simulink model "ElevatorPlant_Storage_A"  (R2015b)
(part 7 of 8)

            (junction 94133) -> Emergency.Doors.Opening2.Button_detection1.BUTTON_CAR.Button_CAR_1 [order 1] : [P1]
            (junction 94133) -> (junction 94134) [order 2]
            (junction 94135) -> (junction 94134)
            (junction 94136) -> (junction 94135)
            (junction 94134) -> (junction 94137)
            (junction 94137) -> Emergency.Doors.Opening2.Button_detection1.BUTTON_CAR.Button_CAR_2 [order 1] : [P2]
            Emergency.Doors.Opening2.Button_detection1.BUTTON_CAR.Button_CAR_2 -> (junction 94138)
            (junction 94138) -> Emergency.Doors.Opening2.Button_detection1.BUTTON_CAR.First_but_2 [order 1] : [FIRST_BUT && not(RPC2)]
            Emergency.Doors.Opening2.Button_detection1.BUTTON_CAR.First_but_2 -> (junction 94139)
            (junction 94137) -> (junction 94140) [order 2]
            (junction 94138) -> (junction 94141) [order 2]
            (junction 94139) -> (junction 94142)
            (junction 94141) -> (junction 94140)
            (junction 94142) -> (junction 94141)
            (junction 94140) -> (junction 94143)
            (junction 94143) -> Emergency.Doors.Opening2.Button_detection1.BUTTON_CAR.Button_CAR_3 [order 1] : [P3]
            Emergency.Doors.Opening2.Button_detection1.BUTTON_CAR.Button_CAR_3 -> (junction 94144)
            (junction 94144) -> Emergency.Doors.Opening2.Button_detection1.BUTTON_CAR.First_but_3 [order 1] : [FIRST_BUT && not(RPC3)]
            Emergency.Doors.Opening2.Button_detection1.BUTTON_CAR.First_but_3 -> (junction 94145)
            (junction 94143) -> (junction 94146) [order 2]
            (junction 94144) -> (junction 94147) [order 2]
            (junction 94145) -> (junction 94148)
            (junction 94147) -> (junction 94146)
            (junction 94148) -> (junction 94147)
          state BUTTON_UP
            state Button_UP_0
              en:
              BUTTON_UP(1)=true;
              BUT_TEMP=0;
              LPS0=true;
              PUSHED=true;
              UPDATE=false;
              IN_LL=false; ET_LL=0;
            state First_but_0
              en:
              BUT_1=BUT_TEMP;
              FIRST_BUT=false;
            state Button_UP_1
              en:
              BUTTON_UP(2)=true;
              BUT_TEMP=1;
              LPS1=true;
              PUSHED=true;
              UPDATE=false;
              IN_LL=false; ET_LL=0;
            state First_but_1
              en:
              BUT_1=BUT_TEMP;
              FIRST_BUT=false;
            state Button_UP_2
              en:
              BUTTON_UP(3)=true;
              BUT_TEMP=2;
              LPS2=true;
              PUSHED=true;
              UPDATE=false;
              IN_LL=false; ET_LL=0;
            state First_but_2
              en:
              BUT_1=BUT_TEMP;
              FIRST_BUT=false;
            (junction 94198) -> Emergency.Doors.Opening2.Button_detection1.BUTTON_UP.Button_UP_0 [order 1] : [PS0]
            Emergency.Doors.Opening2.Button_detection1.BUTTON_UP.Button_UP_0 -> (junction 94199)
            (junction 94199) -> Emergency.Doors.Opening2.Button_detection1.BUTTON_UP.First_but_0 [order 1] : [FIRST_BUT && not(RPC0)]
            Emergency.Doors.Opening2.Button_detection1.BUTTON_UP.First_but_0 -> (junction 94200)
            (default) -> (junction 94198)
            (junction 94198) -> (junction 94203) [order 2]
            (junction 94199) -> (junction 94201) [order 2]
            (junction 94200) -> (junction 94202)
            (junction 94202) -> (junction 94201)
            (junction 94201) -> (junction 94203)
            (junction 94203) -> (junction 94204)
            (junction 94204) -> Emergency.Doors.Opening2.Button_detection1.BUTTON_UP.Button_UP_1 [order 1] : [PS1]
            Emergency.Doors.Opening2.Button_detection1.BUTTON_UP.Button_UP_1 -> (junction 94205)
            (junction 94205) -> Emergency.Doors.Opening2.Button_detection1.BUTTON_UP.First_but_1 [order 1] : [FIRST_BUT && not(RPC1)]
            Emergency.Doors.Opening2.Button_detection1.BUTTON_UP.First_but_1 -> (junction 94206)
            (junction 94204) -> (junction 94207) [order 2]
            (junction 94205) -> (junction 94208) [order 2]
            (junction 94206) -> (junction 94209)
            (junction 94208) -> (junction 94207)
            (junction 94209) -> (junction 94208)
            (junction 94207) -> (junction 94211)
            Emergency.Doors.Opening2.Button_detection1.BUTTON_UP.First_but_2 -> (junction 94210)
            (junction 94210) -> (junction 94215)
            (junction 94211) -> Emergency.Doors.Opening2.Button_detection1.BUTTON_UP.Button_UP_2 [order 1] : [PS2]
            Emergency.Doors.Opening2.Button_detection1.BUTTON_UP.Button_UP_2 -> (junction 94212)
            (junction 94212) -> Emergency.Doors.Opening2.Button_detection1.BUTTON_UP.First_but_2 [order 1] : [FIRST_BUT && not(RPC2)]
            (junction 94211) -> (junction 94213) [order 2]
            (junction 94212) -> (junction 94214) [order 2]
            (junction 94214) -> (junction 94213)
            (junction 94215) -> (junction 94214)
          state Max_Min_assignment
            state Min_but
              en:
              BUTTON=MIN_BUT;
            state Max_but
              en:
              BUTTON=MAX_BUT;
            state First_but
              en:
              BUTTON=BUT_1;
            state Max_but1
              en:
              MAX_BUT=2;
            state Max_but2
              en:
              MAX_BUT=1;
            state Max_but3
              en:
              MAX_BUT=0;
            state Min_but1
              en:
              MIN_BUT=1;
            state Min_but2
              en:
              MIN_BUT=2;
            state Min_but3
              en:
              MIN_BUT=3;
            state MAX
              en:
              MAX_BUT=BUT_TEMP;
            state MIN
              en:
              MIN_BUT=BUT_TEMP;
            state Updating_button_0
              en:
              BUTTON=MAX_BUT;
            state Updating_button_1
              en:
              BUTTON=MIN_BUT;
            (junction 94253) -> Emergency.Doors.Opening2.Button_detection1.Max_Min_assignment.Min_but [order 1] : [(MAX_BUT-FLOOR)>(FLOOR-MIN_BUT)]
            Emergency.Doors.Opening2.Button_detection1.Max_Min_assignment.Min_but -> (junction 94254)
            (junction 94255) -> (junction 94253) [order 1] : [not(FLAG_STOP) && MOTION==2 && FLAG==3]
            (default) -> (junction 94255)
            (junction 94253) -> (junction 94256) [order 2]
            (junction 94254) -> (junction 94257)
            (junction 94255) -> (junction 94258) [order 2]
            (junction 94256) -> Emergency.Doors.Opening2.Button_detection1.Max_Min_assignment.Max_but [order 1] : [(MAX_BUT-FLOOR)<(FLOOR-MIN_BUT)]
            Emergency.Doors.Opening2.Button_detection1.Max_Min_assignment.Max_but -> (junction 94257)
            (junction 94256) -> Emergency.Doors.Opening2.Button_detection1.Max_Min_assignment.First_but [order 2]
            (junction 94257) -> (junction 94260)
            Emergency.Doors.Opening2.Button_detection1.Max_Min_assignment.First_but -> (junction 94259)
            (junction 94259) -> (junction 94258)
            (junction 94260) -> (junction 94259)
            (junction 94258) -> (junction 94261)
            (junction 94262) -> (junction 94263) [order 1] : [MOTION==0]
                | {MOTION=1;
                | UPDATE=true;}
            (junction 94263) -> Emergency.Doors.Opening2.Button_detection1.Max_Min_assignment.Max_but1 [order 1] : [BUTTON_UP(2)]
            Emergency.Doors.Opening2.Button_detection1.Max_Min_assignment.Max_but1 -> (junction 94264)
            (junction 94261) -> (junction 94262) [order 1] : [BUTTON==FLOOR && EXTEND]
                | {EXTEND=false;}
            (junction 94261) -> (junction 94275) [order 2]
            (junction 94262) -> (junction 94267) [order 2]
            (junction 94263) -> (junction 94265) [order 2]
            (junction 94264) -> (junction 94266)
            (junction 94265) -> Emergency.Doors.Opening2.Button_detection1.Max_Min_assignment.Max_but2 [order 1] : [BUTTON_UP(1)]
            Emergency.Doors.Opening2.Button_detection1.Max_Min_assignment.Max_but2 -> (junction 94266)
            (junction 94265) -> Emergency.Doors.Opening2.Button_detection1.Max_Min_assignment.Max_but3 [order 2]
            (junction 94266) -> (junction 94269)
            Emergency.Doors.Opening2.Button_detection1.Max_Min_assignment.Max_but3 -> (junction 94268)
            (junction 94268) -> (junction 94267)
            (junction 94269) -> (junction 94268)
            (junction 94267) -> (junction 94270)
            (junction 94270) -> (junction 94271) [order 1] : [MOTION==1]
                | {MOTION=0;
                | UPDATE=true;}
            (junction 94271) -> Emergency.Doors.Opening2.Button_detection1.Max_Min_assignment.Min_but1 [order 1] : [BUTTON_DOWN(1)]
            Emergency.Doors.Opening2.Button_detection1.Max_Min_assignment.Min_but1 -> (junction 94272)
            (junction 94270) -> (junction 94276) [order 2]
            (junction 94271) -> (junction 94273) [order 2]
            (junction 94272) -> (junction 94274)
            (junction 94273) -> Emergency.Doors.Opening2.Button_detection1.Max_Min_assignment.Min_but2 [order 1] : [BUTTON_DOWN(2)]
            Emergency.Doors.Opening2.Button_detection1.Max_Min_assignment.Min_but2 -> (junction 94274)
            (junction 94273) -> Emergency.Doors.Opening2.Button_detection1.Max_Min_assignment.Min_but3 [order 2]
            (junction 94274) -> (junction 94278)
            Emergency.Doors.Opening2.Button_detection1.Max_Min_assignment.Min_but3 -> (junction 94277)
            (junction 94276) -> (junction 94275)
            (junction 94277) -> (junction 94276)
            (junction 94278) -> (junction 94277)
            (junction 94275) -> (junction 94280)
            Emergency.Doors.Opening2.Button_detection1.Max_Min_assignment.MAX -> (junction 94279)
            (junction 94280) -> (junction 94281) [order 1] : [PUSHED]
            (junction 94281) -> (junction 94282) [order 1] : [not(BUT_TEMP==FLOOR) || not(MOTION==2)]
            (junction 94282) -> Emergency.Doors.Opening2.Button_detection1.Max_Min_assignment.MAX [order 1] : [MAX_BUT<BUT_TEMP && not(UPDATE)]
            (junction 94279) -> (junction 94284)
            (junction 94280) -> (junction 94294) [order 2]
            (junction 94281) -> (junction 94287) [order 2]
            (junction 94282) -> (junction 94283) [order 2]
            (junction 94284) -> (junction 94283)
            (junction 94283) -> (junction 94285)
            (junction 94285) -> Emergency.Doors.Opening2.Button_detection1.Max_Min_assignment.MIN [order 1] : [MIN_BUT>BUT_TEMP && not(UPDATE)]
            Emergency.Doors.Opening2.Button_detection1.Max_Min_assignment.MIN -> (junction 94286)
            (junction 94285) -> (junction 94288) [order 2]
            (junction 94286) -> (junction 94289)
            (junction 94288) -> (junction 94287)
            (junction 94289) -> (junction 94288)
            (junction 94287) -> (junction 94290)
            (junction 94290) -> Emergency.Doors.Opening2.Button_detection1.Max_Min_assignment.Updating_button_0 [order 1] : [MOTION==0]
            Emergency.Doors.Opening2.Button_detection1.Max_Min_assignment.Updating_button_0 -> (junction 94291)
            (junction 94290) -> (junction 94292) [order 2]
            (junction 94291) -> (junction 94293)
            (junction 94292) -> Emergency.Doors.Opening2.Button_detection1.Max_Min_assignment.Updating_button_1 [order 1] : [MOTION==1]
            Emergency.Doors.Opening2.Button_detection1.Max_Min_assignment.Updating_button_1 -> (junction 94293)
            (junction 94292) -> (junction 94295) [order 2]
            (junction 94293) -> (junction 94296)
            (junction 94295) -> (junction 94294)
            (junction 94296) -> (junction 94295)
          state GoTo_PositionControl
            en:
            BUTTON=BUT_TEMP;
            FLAG=2;
          state Emergency
            en:
            FLAG_EMG=true;
            FLAG=4;
          state Timer_EME
            state Set_tmr
              en:
              Q_EME=true;
            state Counting
              en:
              ET_EME= ET_EME + 1;
              Q_EME=false;
            state Set
              en:
              IN_EME=true;
              PT_EME=3;
            (junction 94386) -> Emergency.Doors.Opening2.Button_detection1.Timer_EME.Set_tmr [order 1] : [ET_EME==PT_EME]
            Emergency.Doors.Opening2.Button_detection1.Timer_EME.Set_tmr -> (junction 94387)
            Emergency.Doors.Opening2.Button_detection1.Timer_EME.Counting -> (junction 94386)
            (junction 94386) -> (junction 94387) [order 2]
            (default) -> Emergency.Doors.Opening2.Button_detection1.Timer_EME.Set
            Emergency.Doors.Opening2.Button_detection1.Timer_EME.Set -> (junction 94388)
            (junction 94388) -> Emergency.Doors.Opening2.Button_detection1.Timer_EME.Counting [order 1] : [ET_EME<PT_EME]
            (junction 94388) -> (junction 94387) [order 2]
          state Not_Emergency
            en:
            IN_EME=false;
            ET_EME=0;
          state SwitchingOFF_LEDs
            en:
            LPD3=false;
            LPD2=false;
            LPS2=false;
            LPD1=false;
            LPS1=false;
            LPS0=false;
          (default) -> (junction 93987)
          (junction 93987) -> (junction 93988) [order 1] : [FLAG==1 && not(PUSHED)]
              | {BUTTON=FLOOR;
              | BUT_TEMP=BUTTON;
              | BUT_1=FLOOR;}
          (junction 93988) -> Emergency.Doors.Opening2.Button_detection1.Timer_LL [order 1] : [not(FLAG_STOP)]
          Emergency.Doors.Opening2.Button_detection1.Save_energy -> (junction 93989)
          Emergency.Doors.Opening2.Button_detection1.Timer_LL -> Emergency.Doors.Opening2.Button_detection1.Save_energy
          (junction 93988) -> (junction 93991) [order 2]
          (junction 93987) -> (junction 93990) [order 2]
          (junction 93989) -> (junction 93992)
          (junction 93991) -> (junction 93990)
          (junction 93992) -> (junction 93991)
          (junction 93990) -> Emergency.Doors.Opening2.Button_detection1.BUTTON_CAR
          Emergency.Doors.Opening2.Button_detection1.BUTTON_UP -> Emergency.Doors.Opening2.Button_detection1.BUTTON_DOWN
          Emergency.Doors.Opening2.Button_detection1.BUTTON_DOWN -> Emergency.Doors.Opening2.Button_detection1.Max_Min_assignment
          Emergency.Doors.Opening2.Button_detection1.Max_Min_assignment -> (junction 93993)
          Emergency.Doors.Opening2.Button_detection1.BUTTON_CAR -> Emergency.Doors.Opening2.Button_detection1.BUTTON_UP
          (junction 93993) -> (junction 93995)
          (junction 93995) -> (junction 93994)
          (junction 93994) -> (junction 93997)
          Emergency.Doors.Opening2.Button_detection1.GoTo_PositionControl -> (junction 93996)
          (junction 93997) -> (junction 93998) [order 1] : [FLAG==1]
          (junction 93998) -> Emergency.Doors.Opening2.Button_detection1.GoTo_PositionControl [order 1] : [PUSHED]
          (junction 93996) -> (junction 94000)
          (junction 93997) -> (junction 94008) [order 2]
          (junction 93998) -> (junction 93999) [order 2]
          (junction 94000) -> (junction 93999)
          (junction 93999) -> (junction 94002)
          Emergency.Doors.Opening2.Button_detection1.Emergency -> (junction 94001)
          (junction 94002) -> Emergency.Doors.Opening2.Button_detection1.Timer_EME [order 1] : [STOP]
              | {IN_LL=false; ET_LL=0;FLAG=1;}
          Emergency.Doors.Opening2.Button_detection1.Timer_EME -> (junction 94003)
          (junction 94003) -> Emergency.Doors.Opening2.Button_detection1.Emergency [order 1] : [Q_EME]
          (junction 94001) -> (junction 94005)
          (junction 94002) -> Emergency.Doors.Opening2.Button_detection1.Not_Emergency [order 2]
          (junction 94003) -> (junction 94004) [order 2]
          (junction 94005) -> (junction 94004)
          (junction 94004) -> (junction 94007)
          Emergency.Doors.Opening2.Button_detection1.Not_Emergency -> (junction 94007)
          Emergency.Doors.Opening2.Button_detection1.SwitchingOFF_LEDs -> (junction 94006)
          (junction 94007) -> Emergency.Doors.Opening2.Button_detection1.SwitchingOFF_LEDs [order 1] : [FLAG_STOP && FLAG==2]
          (junction 94006) -> (junction 94010)
          (junction 94007) -> (junction 94009) [order 2]
          (junction 94009) -> (junction 94008)
          (junction 94010) -> (junction 94009)
        state Opening1
          en:AP2=true;
        state Reset
          state Reset_0
            en:
            LPS0=false;
            BUTTON_CAR(1)=false;
            BUTTON_UP(1)=false;
          state Reset_1
            en:
            LPS1=false;
            LPD1=false;
            BUTTON_CAR(2)=false;
            BUTTON_UP(2)=false;
            BUTTON_DOWN(2)=false;
          state Reset_2
            en:
            LPS2=false;
            LPD2=false;
            BUTTON_CAR(3)=false;
            BUTTON_UP(3)=false;
            BUTTON_DOWN(3)=false;
          state Reset_3
            en:
            LPD3=false;
            BUTTON_CAR(4)=false;
            BUTTON_DOWN(4)=false;
          (default) -> (junction 94404)
          (junction 94404) -> Emergency.Doors.Opening2.Reset.Reset_0 [order 1] : [FLOOR==0]
          Emergency.Doors.Opening2.Reset.Reset_0 -> (junction 94405)
          (junction 94404) -> (junction 94406) [order 2]
          (junction 94405) -> (junction 94407)
          (junction 94406) -> Emergency.Doors.Opening2.Reset.Reset_1 [order 1] : [FLOOR==1]
          Emergency.Doors.Opening2.Reset.Reset_1 -> (junction 94407)
          (junction 94406) -> (junction 94408) [order 2]
          (junction 94407) -> (junction 94409)
          (junction 94408) -> Emergency.Doors.Opening2.Reset.Reset_2 [order 1] : [FLOOR==2]
          Emergency.Doors.Opening2.Reset.Reset_2 -> (junction 94409)
          (junction 94408) -> (junction 94410) [order 2]
          (junction 94409) -> (junction 94411)
          (junction 94410) -> Emergency.Doors.Opening2.Reset.Reset_3 [order 1] : [FLOOR==3]
          Emergency.Doors.Opening2.Reset.Reset_3 -> (junction 94411)
          (junction 94410) -> (junction 94412) [order 2]
          (junction 94411) -> (junction 94413)
          (junction 94413) -> (junction 94412)
        state Stop_Opening1
          en: AP2=false;
          FLAG_OD=true;
          IN_cl=false;
          ET_cl=0;
        (junction 93401) -> (junction 93402)
        (junction 93402) -> (junction 93403) [order 1] : [not(OBS) ]
        (junction 93405) -> Emergency.Doors.Opening2.Opening [order 1] : [not(PA2)]
        (junction 93403) -> (junction 93404) [order 2]
        (junction 93404) -> Emergency.Doors.Opening2.Timer_open
        Emergency.Doors.Opening2.Timer_open -> (junction 93405)
        (default) -> Emergency.Doors.Opening2.People_IN
        (junction 93402) -> (junction 93406) [order 2]
        (junction 93403) -> Emergency.Doors.Opening2.Button_detection [order 1] : [not(FLAG==4)]
        (junction 93408) -> (junction 93404)
        (junction 93410) -> (junction 93401)
        (junction 93405) -> Emergency.Doors.Opening2.Stop_Opening [order 2]
        Emergency.Doors.Opening2.People_IN -> Emergency.Doors.Opening2.People_OUT
        Emergency.Doors.Opening2.Opening -> (junction 93415)
        (junction 93406) -> (junction 93407) [order 2]
        (junction 93406) -> Emergency.Doors.Opening2.Button_detection1 [order 1] : [not(FLAG==4)]
        (junction 93407) -> (junction 93412)
        Emergency.Doors.Opening2.Button_detection -> (junction 93408)
        Emergency.Doors.Opening2.People_OUT -> (junction 93409)
        Emergency.Doors.Opening2.Button_detection1 -> (junction 93411)
        (junction 93412) -> (junction 93411)
        (junction 93409) -> (junction 93410) [order 2]
        (junction 93409) -> Emergency.Doors.Opening2.Reset [order 1] : [not(FLAG==4)]
        (junction 93411) -> (junction 93413)
        (junction 93419) -> (junction 93410)
        Emergency.Doors.Opening2.Stop_Opening -> (junction 93414)
        (junction 93413) -> Emergency.Doors.Opening2.Opening1 [order 1] : [not(PA2)]
        (junction 93413) -> Emergency.Doors.Opening2.Stop_Opening1 [order 2]
        (junction 93415) -> (junction 93414)
        (junction 93414) -> (junction 93417)
        Emergency.Doors.Opening2.Opening1 -> (junction 93416)
        Emergency.Doors.Opening2.Reset -> (junction 93418)
        Emergency.Doors.Opening2.Stop_Opening1 -> (junction 93416)
        (junction 93416) -> (junction 93417)
        (junction 93418) -> (junction 93419)
      state FLOOR_3
        en: CP3=false;
      state Opening3
        state Opening
          en:AP3=Q_op;
        state People_IN
          state Check_People_IN
            en:
            COUNTER_IN=false;
          state People_KID_IN
            en:
            WEIGHT=WEIGHT+30;
            KIDS=KIDS+1;
          state People_WOMAN_IN
            en:
            WEIGHT=WEIGHT+55;
            WOMEN=WOMEN+1;
          state People_MAN_IN
            en:
            WEIGHT=WEIGHT+75;
            MEN=MEN+1;
          state People_FATGUY_IN
            en:
            WEIGHT=WEIGHT+100;
            FATGUYS=FATGUYS+1;
          state Re_Ready_IN
            en:
            COUNTER_IN=true;
          (default) -> (junction 94494)
          (junction 94494) -> Emergency.Doors.Opening3.People_IN.Check_People_IN [order 1] : [COUNTER_IN]
          Emergency.Doors.Opening3.People_IN.Check_People_IN -> (junction 94495)
          (junction 94495) -> Emergency.Doors.Opening3.People_IN.People_KID_IN [order 1] : [KID_IN]
          Emergency.Doors.Opening3.People_IN.People_KID_IN -> (junction 94496)
          (junction 94494) -> (junction 94503) [order 2]
          (junction 94495) -> (junction 94497) [order 2]
          (junction 94496) -> (junction 94498)
          (junction 94497) -> Emergency.Doors.Opening3.People_IN.People_WOMAN_IN [order 1] : [WOMAN_IN]
          Emergency.Doors.Opening3.People_IN.People_WOMAN_IN -> (junction 94498)
          (junction 94497) -> (junction 94499) [order 2]
          (junction 94498) -> (junction 94500)
          (junction 94499) -> Emergency.Doors.Opening3.People_IN.People_MAN_IN [order 1] : [MAN_IN]
          Emergency.Doors.Opening3.People_IN.People_MAN_IN -> (junction 94500)
          (junction 94499) -> (junction 94501) [order 2]
          (junction 94500) -> (junction 94502)
          (junction 94501) -> Emergency.Doors.Opening3.People_IN.People_FATGUY_IN [order 1] : [FATGUY_IN]
          Emergency.Doors.Opening3.People_IN.People_FATGUY_IN -> (junction 94502)
          (junction 94501) -> (junction 94504) [order 2]
          (junction 94502) -> (junction 94505)
          (junction 94504) -> (junction 94503)
          (junction 94505) -> (junction 94504)
          (junction 94503) -> (junction 94506)
          (junction 94506) -> Emergency.Doors.Opening3.People_IN.Re_Ready_IN [order 1] : [not(KID_IN|| WOMAN_IN || MAN_IN || FATGUY_IN)]
          (junction 94506) -> (junction 94507) [order 2]
          Emergency.Doors.Opening3.People_IN.Re_Ready_IN -> (junction 94508)
          (junction 94508) -> (junction 94507)
        state Timer_open
          state Set_tmr
            en: Q_op=true;
          state Set
            en:PT_op=2;
            IN_op=true;
          state Counting
            en:ET_op = ET_op + 1;
            Q_op=false;
          (junction 94543) -> Emergency.Doors.Opening3.Timer_open.Set_tmr [order 1] : [ET_op==PT_op]
          Emergency.Doors.Opening3.Timer_open.Set_tmr -> (junction 94544)
          (default) -> Emergency.Doors.Opening3.Timer_open.Set
          Emergency.Doors.Opening3.Timer_open.Counting -> (junction 94543)
          (junction 94543) -> (junction 94544) [order 2]
          Emergency.Doors.Opening3.Timer_open.Set -> (junction 94545)
          (junction 94545) -> Emergency.Doors.Opening3.Timer_open.Counting [order 1] : [ET_op<PT_op]
          (junction 94545) -> (junction 94544) [order 2]
        state Stop_Opening
          en:AP3=false;
          FLAG_OD=true;
          OBS=true;
          IN_op=false;
          ET_op=0;
        state People_OUT
          state Check_People_OUT
            en:
            COUNTER_OUT=false;
          state People_KID_OUT
            en:
            WEIGHT=WEIGHT-30;
            KIDS=KIDS-1;
          state People_WOMAN_OUT
            en:
            WEIGHT=WEIGHT-55;
            WOMEN=WOMEN-1;
          state People_MAN_OUT
            en:
            WEIGHT=WEIGHT-75;
            MEN=MEN-1;
          state People_FATGUY_OUT
            en:
            WEIGHT=WEIGHT-100;
            FATGUYS=FATGUYS-1;
          state Re_Ready_OUT
            en:
            COUNTER_OUT=true;
          (default) -> (junction 94559)
          (junction 94559) -> Emergency.Doors.Opening3.People_OUT.Check_People_OUT [order 1] : [COUNTER_OUT]
          Emergency.Doors.Opening3.People_OUT.Check_People_OUT -> (junction 94560)
          (junction 94560) -> Emergency.Doors.Opening3.People_OUT.People_KID_OUT [order 1] : [KID_OUT && KIDS>0 ]
          Emergency.Doors.Opening3.People_OUT.People_KID_OUT -> (junction 94561)
          (junction 94559) -> (junction 94568) [order 2]
          (junction 94560) -> (junction 94562) [order 2]
          (junction 94561) -> (junction 94563)
          (junction 94562) -> Emergency.Doors.Opening3.People_OUT.People_WOMAN_OUT [order 1] : [WOMAN_OUT && WOMEN>0]
          Emergency.Doors.Opening3.People_OUT.People_WOMAN_OUT -> (junction 94563)
          (junction 94563) -> (junction 94565)
          (junction 94562) -> (junction 94564) [order 2]
          (junction 94564) -> Emergency.Doors.Opening3.People_OUT.People_MAN_OUT [order 1] : [MAN_OUT && MEN>0]
          Emergency.Doors.Opening3.People_OUT.People_MAN_OUT -> (junction 94565)
          (junction 94564) -> (junction 94566) [order 2]
          (junction 94565) -> (junction 94567)
          (junction 94566) -> Emergency.Doors.Opening3.People_OUT.People_FATGUY_OUT [order 1] : [FATGUY_OUT && FATGUYS>0]
          Emergency.Doors.Opening3.People_OUT.People_FATGUY_OUT -> (junction 94567)
          (junction 94566) -> (junction 94569) [order 2]
          (junction 94567) -> (junction 94570)
          (junction 94569) -> (junction 94568)
          (junction 94570) -> (junction 94569)
          (junction 94568) -> (junction 94571)
          (junction 94571) -> Emergency.Doors.Opening3.People_OUT.Re_Ready_OUT [order 1] : [not(KID_OUT || WOMAN_OUT || MAN_OUT || FATGUY_OUT)]
          (junction 94571) -> (junction 94572) [order 2]
          Emergency.Doors.Opening3.People_OUT.Re_Ready_OUT -> (junction 94573)
          (junction 94573) -> (junction 94572)
        state Button_detection
          state Save_energy
            en:
            LL=not(Q_LL);
          state Timer_LL
            state Set_tmr
              en:
              Q_LL=true;
            state Counting
              en:
              ET_LL= ET_LL + 1;
              Q_LL=false;
            state Set
              en:
              IN_LL=true;
              PT_LL=10;
            (junction 94676) -> Emergency.Doors.Opening3.Button_detection.Timer_LL.Set_tmr [order 1] : [ET_LL==PT_LL]
            Emergency.Doors.Opening3.Button_detection.Timer_LL.Set_tmr -> (junction 94677)
            Emergency.Doors.Opening3.Button_detection.Timer_LL.Counting -> (junction 94676)
            (junction 94676) -> (junction 94677) [order 2]
            (default) -> Emergency.Doors.Opening3.Button_detection.Timer_LL.Set
            Emergency.Doors.Opening3.Button_detection.Timer_LL.Set -> (junction 94678)
            (junction 94678) -> Emergency.Doors.Opening3.Button_detection.Timer_LL.Counting [order 1] : [ET_LL<PT_LL]
            (junction 94678) -> (junction 94677) [order 2]
          state BUTTON_DOWN
            state Button_DOWN_1
              en:
              BUTTON_DOWN(2)=true;
              BUT_TEMP=1;
              LPD1=true;
              PUSHED=true;
              UPDATE=false;
              IN_LL=false; ET_LL=0;
            state First_but_1
              en:
              BUT_1=BUT_TEMP;
              FIRST_BUT=false;
            state Button_DOWN_2
              en:
              BUTTON_DOWN(3)=true;
              BUT_TEMP=2;
              LPD2=true;
              PUSHED=true;
              UPDATE=false;
              IN_LL=false; ET_LL=0;
            state First_but_2
              en:
              BUT_1=BUT_TEMP;
              FIRST_BUT=false;
            state Button_DOWN_3
              en:
              BUTTON_DOWN(4)=true;
              BUT_TEMP=3;
              LPD3=true;
              PUSHED=true;
              UPDATE=false;
              IN_LL=false; ET_LL=0;
            state First_but_3
              en:
              BUT_1=BUT_TEMP;
              FIRST_BUT=false;
            (default) -> (junction 94691)
            (junction 94691) -> Emergency.Doors.Opening3.Button_detection.BUTTON_DOWN.Button_DOWN_1 [order 1] : [PD1]
            Emergency.Doors.Opening3.Button_detection.BUTTON_DOWN.Button_DOWN_1 -> (junction 94692)
            (junction 94692) -> Emergency.Doors.Opening3.Button_detection.BUTTON_DOWN.First_but_1 [order 1] : [FIRST_BUT && not(RPC1)]
            Emergency.Doors.Opening3.Button_detection.BUTTON_DOWN.First_but_1 -> (junction 94693)
            (junction 94691) -> (junction 94694) [order 2]
            (junction 94692) -> (junction 94695) [order 2]
            (junction 94693) -> (junction 94696)
            (junction 94695) -> (junction 94694)
            (junction 94696) -> (junction 94695)
            (junction 94694) -> (junction 94697)
            (junction 94697) -> Emergency.Doors.Opening3.Button_detection.BUTTON_DOWN.Button_DOWN_2 [order 1] : [PD2]
            Emergency.Doors.Opening3.Button_detection.BUTTON_DOWN.Button_DOWN_2 -> (junction 94698)
            (junction 94698) -> Emergency.Doors.Opening3.Button_detection.BUTTON_DOWN.First_but_2 [order 1] : [FIRST_BUT && not(RPC2)]
            Emergency.Doors.Opening3.Button_detection.BUTTON_DOWN.First_but_2 -> (junction 94699)
            (junction 94697) -> (junction 94700) [order 2]
            (junction 94698) -> (junction 94701) [order 2]
            (junction 94699) -> (junction 94702)
            (junction 94701) -> (junction 94700)
            (junction 94702) -> (junction 94701)
            (junction 94700) -> (junction 94703)
            (junction 94703) -> Emergency.Doors.Opening3.Button_detection.BUTTON_DOWN.Button_DOWN_3 [order 1] : [PD3]
            Emergency.Doors.Opening3.Button_detection.BUTTON_DOWN.Button_DOWN_3 -> (junction 94704)
            (junction 94704) -> Emergency.Doors.Opening3.Button_detection.BUTTON_DOWN.First_but_3 [order 1] : [FIRST_BUT && not(RPC3)]
            Emergency.Doors.Opening3.Button_detection.BUTTON_DOWN.First_but_3 -> (junction 94705)
            (junction 94703) -> (junction 94706) [order 2]
            (junction 94704) -> (junction 94707) [order 2]
            (junction 94705) -> (junction 94708)
            (junction 94707) -> (junction 94706)
            (junction 94708) -> (junction 94707)
          state BUTTON_CAR
            state Button_CAR_0
              en:
              BUTTON_CAR(1)=true;
              BUT_TEMP=0;
              LPC0=true;
              PUSHED=true;
              UPDATE=false;
              IN_LL=false; ET_LL=0;
            state First_but_0
              en:
              BUT_1=BUT_TEMP;
              FIRST_BUT=false;
            state Button_CAR_1
              en:
              BUTTON_CAR(2)=true;
              BUT_TEMP=1;
              LPC1=true;
              PUSHED=true;
              UPDATE=false;
              IN_LL=false; ET_LL=0;
            state First_but_1
              en:
              BUT_1=BUT_TEMP;
              FIRST_BUT=false;
            state Button_CAR_2
              en:
              BUTTON_CAR(3)=true;
              BUT_TEMP=2;
              LPC2=true;
              PUSHED=true;
              UPDATE=false;
              IN_LL=false; ET_LL=0;
            state First_but_2
              en:
              BUT_1=BUT_TEMP;
              FIRST_BUT=false;
            state Button_CAR_3
              en:
              BUTTON_CAR(4)=true;
              BUT_TEMP=3;
              LPC3=true;
              PUSHED=true;
              UPDATE=false;
              IN_LL=false; ET_LL=0;
            state First_but_3
              en:
              BUT_1=BUT_TEMP;
              FIRST_BUT=false;
            (default) -> (junction 94746)
            (junction 94746) -> Emergency.Doors.Opening3.Button_detection.BUTTON_CAR.Button_CAR_0 [order 1] : [P0]
            Emergency.Doors.Opening3.Button_detection.BUTTON_CAR.Button_CAR_0 -> (junction 94747)
            (junction 94747) -> Emergency.Doors.Opening3.Button_detection.BUTTON_CAR.First_but_0 [order 1] : [FIRST_BUT && not(RPC0)]
            Emergency.Doors.Opening3.Button_detection.BUTTON_CAR.First_but_0 -> (junction 94748)
            (junction 94746) -> (junction 94749) [order 2]
            (junction 94747) -> (junction 94750) [order 2]
            (junction 94748) -> (junction 94751)
            (junction 94750) -> (junction 94749)
            (junction 94751) -> (junction 94750)
            (junction 94749) -> (junction 94754)
            Emergency.Doors.Opening3.Button_detection.BUTTON_CAR.Button_CAR_1 -> (junction 94752)
            (junction 94752) -> Emergency.Doors.Opening3.Button_detection.BUTTON_CAR.First_but_1 [order 1] : [FIRST_BUT && not(RPC1)]
            Emergency.Doors.Opening3.Button_detection.BUTTON_CAR.First_but_1 -> (junction 94753)
            (junction 94752) -> (junction 94756) [order 2]
            (junction 94753) -> (junction 94757)
            (junction 94754) -> Emergency.Doors.Opening3.Button_detection.BUTTON_CAR.Button_CAR_1 [order 1] : [P1]
            (junction 94754) -> (junction 94755) [order 2]
            (junction 94756) -> (junction 94755)
            (junction 94757) -> (junction 94756)
            (junction 94755) -> (junction 94758)
            (junction 94758) -> Emergency.Doors.Opening3.Button_detection.BUTTON_CAR.Button_CAR_2 [order 1] : [P2]
            Emergency.Doors.Opening3.Button_detection.BUTTON_CAR.Button_CAR_2 -> (junction 94759)
            (junction 94759) -> Emergency.Doors.Opening3.Button_detection.BUTTON_CAR.First_but_2 [order 1] : [FIRST_BUT && not(RPC2)]
            Emergency.Doors.Opening3.Button_detection.BUTTON_CAR.First_but_2 -> (junction 94760)
            (junction 94758) -> (junction 94761) [order 2]
            (junction 94759) -> (junction 94762) [order 2]
            (junction 94760) -> (junction 94763)
            (junction 94762) -> (junction 94761)
            (junction 94763) -> (junction 94762)
            (junction 94761) -> (junction 94764)
            (junction 94764) -> Emergency.Doors.Opening3.Button_detection.BUTTON_CAR.Button_CAR_3 [order 1] : [P3]
            Emergency.Doors.Opening3.Button_detection.BUTTON_CAR.Button_CAR_3 -> (junction 94765)
            (junction 94765) -> Emergency.Doors.Opening3.Button_detection.BUTTON_CAR.First_but_3 [order 1] : [FIRST_BUT && not(RPC3)]
            Emergency.Doors.Opening3.Button_detection.BUTTON_CAR.First_but_3 -> (junction 94766)
            (junction 94764) -> (junction 94767) [order 2]
            (junction 94765) -> (junction 94768) [order 2]
            (junction 94766) -> (junction 94769)
            (junction 94768) -> (junction 94767)
            (junction 94769) -> (junction 94768)
          state BUTTON_UP
            state Button_UP_0
              en:
              BUTTON_UP(1)=true;
              BUT_TEMP=0;
              LPS0=true;
              PUSHED=true;
              UPDATE=false;
              IN_LL=false; ET_LL=0;
            state First_but_0
              en:
              BUT_1=BUT_TEMP;
              FIRST_BUT=false;
            state Button_UP_1
              en:
              BUTTON_UP(2)=true;
              BUT_TEMP=1;
              LPS1=true;
              PUSHED=true;
              UPDATE=false;
              IN_LL=false; ET_LL=0;
            state First_but_1
              en:
              BUT_1=BUT_TEMP;
              FIRST_BUT=false;
            state Button_UP_2
              en:
              BUTTON_UP(3)=true;
              BUT_TEMP=2;
              LPS2=true;
              PUSHED=true;
              UPDATE=false;
              IN_LL=false; ET_LL=0;
            state First_but_2
              en:
              BUT_1=BUT_TEMP;
              FIRST_BUT=false;
            (junction 94819) -> Emergency.Doors.Opening3.Button_detection.BUTTON_UP.Button_UP_0 [order 1] : [PS0]
            Emergency.Doors.Opening3.Button_detection.BUTTON_UP.Button_UP_0 -> (junction 94820)
            (junction 94820) -> Emergency.Doors.Opening3.Button_detection.BUTTON_UP.First_but_0 [order 1] : [FIRST_BUT && not(RPC0)]
            Emergency.Doors.Opening3.Button_detection.BUTTON_UP.First_but_0 -> (junction 94821)
            (default) -> (junction 94819)
            (junction 94819) -> (junction 94824) [order 2]
            (junction 94820) -> (junction 94822) [order 2]
            (junction 94821) -> (junction 94823)
            (junction 94823) -> (junction 94822)
            (junction 94822) -> (junction 94824)
            (junction 94824) -> (junction 94825)
            (junction 94825) -> Emergency.Doors.Opening3.Button_detection.BUTTON_UP.Button_UP_1 [order 1] : [PS1]
            Emergency.Doors.Opening3.Button_detection.BUTTON_UP.Button_UP_1 -> (junction 94826)
            (junction 94826) -> Emergency.Doors.Opening3.Button_detection.BUTTON_UP.First_but_1 [order 1] : [FIRST_BUT && not(RPC1)]
            Emergency.Doors.Opening3.Button_detection.BUTTON_UP.First_but_1 -> (junction 94827)
            (junction 94825) -> (junction 94828) [order 2]
            (junction 94826) -> (junction 94829) [order 2]
            (junction 94827) -> (junction 94830)
            (junction 94829) -> (junction 94828)
            (junction 94830) -> (junction 94829)
            (junction 94828) -> (junction 94832)
            Emergency.Doors.Opening3.Button_detection.BUTTON_UP.First_but_2 -> (junction 94831)
            (junction 94831) -> (junction 94836)
            (junction 94832) -> Emergency.Doors.Opening3.Button_detection.BUTTON_UP.Button_UP_2 [order 1] : [PS2]
            Emergency.Doors.Opening3.Button_detection.BUTTON_UP.Button_UP_2 -> (junction 94833)
            (junction 94833) -> Emergency.Doors.Opening3.Button_detection.BUTTON_UP.First_but_2 [order 1] : [FIRST_BUT && not(RPC2)]
            (junction 94832) -> (junction 94834) [order 2]
            (junction 94833) -> (junction 94835) [order 2]
            (junction 94835) -> (junction 94834)
            (junction 94836) -> (junction 94835)
          state Max_Min_assignment
            state Min_but
              en:
              BUTTON=MIN_BUT;
            state Max_but
              en:
              BUTTON=MAX_BUT;
            state First_but
              en:
              BUTTON=BUT_1;
            state Max_but1
              en:
              MAX_BUT=2;
            state Max_but2
              en:
              MAX_BUT=1;
            state Max_but3
              en:
              MAX_BUT=0;
            state Min_but1
              en:
              MIN_BUT=1;
            state Min_but2
              en:
              MIN_BUT=2;
            state Min_but3
              en:
              MIN_BUT=3;
            state MAX
              en:
              MAX_BUT=BUT_TEMP;
            state MIN
              en:
              MIN_BUT=BUT_TEMP;
            state Updating_button_0
              en:
              BUTTON=MAX_BUT;
            state Updating_button_1
              en:
              BUTTON=MIN_BUT;
            (junction 94874) -> Emergency.Doors.Opening3.Button_detection.Max_Min_assignment.Min_but [order 1] : [(MAX_BUT-FLOOR)>(FLOOR-MIN_BUT)]
            Emergency.Doors.Opening3.Button_detection.Max_Min_assignment.Min_but -> (junction 94875)
            (junction 94876) -> (junction 94874) [order 1] : [not(FLAG_STOP) && MOTION==2 && FLAG==3]
            (default) -> (junction 94876)
            (junction 94874) -> (junction 94877) [order 2]
            (junction 94875) -> (junction 94878)
            (junction 94876) -> (junction 94879) [order 2]
            (junction 94877) -> Emergency.Doors.Opening3.Button_detection.Max_Min_assignment.Max_but [order 1] : [(MAX_BUT-FLOOR)<(FLOOR-MIN_BUT)]
            Emergency.Doors.Opening3.Button_detection.Max_Min_assignment.Max_but -> (junction 94878)
            (junction 94877) -> Emergency.Doors.Opening3.Button_detection.Max_Min_assignment.First_but [order 2]
            (junction 94878) -> (junction 94881)
            Emergency.Doors.Opening3.Button_detection.Max_Min_assignment.First_but -> (junction 94880)
            (junction 94880) -> (junction 94879)
            (junction 94881) -> (junction 94880)
            (junction 94879) -> (junction 94882)
            (junction 94883) -> (junction 94884) [order 1] : [MOTION==0]
                | {MOTION=1;
                | UPDATE=true;}
            (junction 94884) -> Emergency.Doors.Opening3.Button_detection.Max_Min_assignment.Max_but1 [order 1] : [BUTTON_UP(2)]
            Emergency.Doors.Opening3.Button_detection.Max_Min_assignment.Max_but1 -> (junction 94885)
            (junction 94882) -> (junction 94883) [order 1] : [BUTTON==FLOOR && EXTEND]
                | {EXTEND=false;}
            (junction 94882) -> (junction 94896) [order 2]
            (junction 94883) -> (junction 94888) [order 2]
            (junction 94884) -> (junction 94886) [order 2]
            (junction 94885) -> (junction 94887)
            (junction 94886) -> Emergency.Doors.Opening3.Button_detection.Max_Min_assignment.Max_but2 [order 1] : [BUTTON_UP(1)]
            Emergency.Doors.Opening3.Button_detection.Max_Min_assignment.Max_but2 -> (junction 94887)
            (junction 94886) -> Emergency.Doors.Opening3.Button_detection.Max_Min_assignment.Max_but3 [order 2]
            (junction 94887) -> (junction 94890)
            Emergency.Doors.Opening3.Button_detection.Max_Min_assignment.Max_but3 -> (junction 94889)
            (junction 94889) -> (junction 94888)
            (junction 94890) -> (junction 94889)
            (junction 94888) -> (junction 94891)
            (junction 94891) -> (junction 94892) [order 1] : [MOTION==1]
                | {MOTION=0;
                | UPDATE=true;}
            (junction 94892) -> Emergency.Doors.Opening3.Button_detection.Max_Min_assignment.Min_but1 [order 1] : [BUTTON_DOWN(1)]
            Emergency.Doors.Opening3.Button_detection.Max_Min_assignment.Min_but1 -> (junction 94893)
            (junction 94891) -> (junction 94897) [order 2]
            (junction 94892) -> (junction 94894) [order 2]
            (junction 94893) -> (junction 94895)
            (junction 94894) -> Emergency.Doors.Opening3.Button_detection.Max_Min_assignment.Min_but2 [order 1] : [BUTTON_DOWN(2)]
            Emergency.Doors.Opening3.Button_detection.Max_Min_assignment.Min_but2 -> (junction 94895)
            (junction 94894) -> Emergency.Doors.Opening3.Button_detection.Max_Min_assignment.Min_but3 [order 2]
            (junction 94895) -> (junction 94899)
            Emergency.Doors.Opening3.Button_detection.Max_Min_assignment.Min_but3 -> (junction 94898)
            (junction 94897) -> (junction 94896)
            (junction 94898) -> (junction 94897)
            (junction 94899) -> (junction 94898)
            (junction 94896) -> (junction 94901)
            Emergency.Doors.Opening3.Button_detection.Max_Min_assignment.MAX -> (junction 94900)
            (junction 94901) -> (junction 94902) [order 1] : [PUSHED]
            (junction 94902) -> (junction 94903) [order 1] : [not(BUT_TEMP==FLOOR) || not(MOTION==2)]
            (junction 94903) -> Emergency.Doors.Opening3.Button_detection.Max_Min_assignment.MAX [order 1] : [MAX_BUT<BUT_TEMP && not(UPDATE)]
            (junction 94900) -> (junction 94905)
            (junction 94901) -> (junction 94915) [order 2]
            (junction 94902) -> (junction 94908) [order 2]
            (junction 94903) -> (junction 94904) [order 2]
            (junction 94905) -> (junction 94904)
            (junction 94904) -> (junction 94906)
            (junction 94906) -> Emergency.Doors.Opening3.Button_detection.Max_Min_assignment.MIN [order 1] : [MIN_BUT>BUT_TEMP && not(UPDATE)]
            Emergency.Doors.Opening3.Button_detection.Max_Min_assignment.MIN -> (junction 94907)
            (junction 94906) -> (junction 94909) [order 2]
            (junction 94907) -> (junction 94910)
            (junction 94909) -> (junction 94908)
            (junction 94910) -> (junction 94909)
            (junction 94908) -> (junction 94911)
            (junction 94911) -> Emergency.Doors.Opening3.Button_detection.Max_Min_assignment.Updating_button_0 [order 1] : [MOTION==0]
            Emergency.Doors.Opening3.Button_detection.Max_Min_assignment.Updating_button_0 -> (junction 94912)
            (junction 94911) -> (junction 94913) [order 2]
            (junction 94912) -> (junction 94914)
            (junction 94913) -> Emergency.Doors.Opening3.Button_detection.Max_Min_assignment.Updating_button_1 [order 1] : [MOTION==1]
            Emergency.Doors.Opening3.Button_detection.Max_Min_assignment.Updating_button_1 -> (junction 94914)
            (junction 94913) -> (junction 94916) [order 2]
            (junction 94914) -> (junction 94917)
            (junction 94916) -> (junction 94915)
            (junction 94917) -> (junction 94916)
          state GoTo_PositionControl
            en:
            BUTTON=BUT_TEMP;
            FLAG=2;
          state Emergency
            en:
            FLAG_EMG=true;
            FLAG=4;
          state Timer_EME
            state Set_tmr
              en:
              Q_EME=true;
            state Counting
              en:
              ET_EME= ET_EME + 1;
              Q_EME=false;
            state Set
              en:
              IN_EME=true;
              PT_EME=3;
            (junction 95007) -> Emergency.Doors.Opening3.Button_detection.Timer_EME.Set_tmr [order 1] : [ET_EME==PT_EME]
            Emergency.Doors.Opening3.Button_detection.Timer_EME.Set_tmr -> (junction 95008)
            Emergency.Doors.Opening3.Button_detection.Timer_EME.Counting -> (junction 95007)
            (junction 95007) -> (junction 95008) [order 2]
            (default) -> Emergency.Doors.Opening3.Button_detection.Timer_EME.Set
            Emergency.Doors.Opening3.Button_detection.Timer_EME.Set -> (junction 95009)
            (junction 95009) -> Emergency.Doors.Opening3.Button_detection.Timer_EME.Counting [order 1] : [ET_EME<PT_EME]
            (junction 95009) -> (junction 95008) [order 2]
          state Not_Emergency
            en:
            IN_EME=false;
            ET_EME=0;
          state SwitchingOFF_LEDs
            en:
            LPD3=false;
            LPD2=false;
            LPS2=false;
            LPD1=false;
            LPS1=false;
            LPS0=false;
          (default) -> (junction 94608)
          (junction 94608) -> (junction 94609) [order 1] : [FLAG==1 && not(PUSHED)]
              | {BUTTON=FLOOR;
              | BUT_TEMP=BUTTON;
              | BUT_1=FLOOR;}
          (junction 94609) -> Emergency.Doors.Opening3.Button_detection.Timer_LL [order 1] : [not(FLAG_STOP)]
          Emergency.Doors.Opening3.Button_detection.Timer_LL -> Emergency.Doors.Opening3.Button_detection.Save_energy
          Emergency.Doors.Opening3.Button_detection.Save_energy -> (junction 94610)
          (junction 94608) -> (junction 94611) [order 2]
          (junction 94609) -> (junction 94612) [order 2]
          (junction 94610) -> (junction 94613)
          (junction 94612) -> (junction 94611)
          (junction 94613) -> (junction 94612)
          (junction 94611) -> Emergency.Doors.Opening3.Button_detection.BUTTON_CAR
          Emergency.Doors.Opening3.Button_detection.BUTTON_UP -> Emergency.Doors.Opening3.Button_detection.BUTTON_DOWN
          Emergency.Doors.Opening3.Button_detection.BUTTON_DOWN -> Emergency.Doors.Opening3.Button_detection.Max_Min_assignment
          Emergency.Doors.Opening3.Button_detection.Max_Min_assignment -> (junction 94614)
          Emergency.Doors.Opening3.Button_detection.BUTTON_CAR -> Emergency.Doors.Opening3.Button_detection.BUTTON_UP
          (junction 94614) -> (junction 94616)
          (junction 94616) -> (junction 94615)
          (junction 94615) -> (junction 94617)
          (junction 94617) -> (junction 94618) [order 1] : [FLAG==1]
          (junction 94618) -> Emergency.Doors.Opening3.Button_detection.GoTo_PositionControl [order 1] : [PUSHED]
          Emergency.Doors.Opening3.Button_detection.GoTo_PositionControl -> (junction 94619)
          (junction 94617) -> (junction 94629) [order 2]
          (junction 94618) -> (junction 94620) [order 2]
          (junction 94619) -> (junction 94621)
          (junction 94621) -> (junction 94620)
          (junction 94620) -> (junction 94623)
          Emergency.Doors.Opening3.Button_detection.Emergency -> (junction 94622)
          (junction 94623) -> Emergency.Doors.Opening3.Button_detection.Timer_EME [order 1] : [STOP]
              | {IN_LL=false; ET_LL=0;FLAG=1;}
          Emergency.Doors.Opening3.Button_detection.Timer_EME -> (junction 94624)
          (junction 94624) -> Emergency.Doors.Opening3.Button_detection.Emergency [order 1] : [Q_EME]
          (junction 94622) -> (junction 94626)
          (junction 94623) -> Emergency.Doors.Opening3.Button_detection.Not_Emergency [order 2]
          (junction 94624) -> (junction 94625) [order 2]
          (junction 94626) -> (junction 94625)
          (junction 94625) -> (junction 94628)
          Emergency.Doors.Opening3.Button_detection.Not_Emergency -> (junction 94628)
          Emergency.Doors.Opening3.Button_detection.SwitchingOFF_LEDs -> (junction 94627)
          (junction 94628) -> Emergency.Doors.Opening3.Button_detection.SwitchingOFF_LEDs [order 1] : [FLAG_STOP && FLAG==2]
          (junction 94627) -> (junction 94631)
          (junction 94628) -> (junction 94630) [order 2]
          (junction 94630) -> (junction 94629)
          (junction 94631) -> (junction 94630)
        state Button_detection1
          state Save_energy
            en:
            LL=not(Q_LL);
          state Timer_LL
            state Set_tmr
              en:
              Q_LL=true;
            state Counting
              en:
              ET_LL= ET_LL + 1;
              Q_LL=false;
            state Set
              en:
              IN_LL=true;
              PT_LL=10;
            (junction 95092) -> Emergency.Doors.Opening3.Button_detection1.Timer_LL.Set_tmr [order 1] : [ET_LL==PT_LL]
            Emergency.Doors.Opening3.Button_detection1.Timer_LL.Set_tmr -> (junction 95093)
            Emergency.Doors.Opening3.Button_detection1.Timer_LL.Counting -> (junction 95092)
            (junction 95092) -> (junction 95093) [order 2]
            (default) -> Emergency.Doors.Opening3.Button_detection1.Timer_LL.Set
            Emergency.Doors.Opening3.Button_detection1.Timer_LL.Set -> (junction 95094)
            (junction 95094) -> Emergency.Doors.Opening3.Button_detection1.Timer_LL.Counting [order 1] : [ET_LL<PT_LL]
            (junction 95094) -> (junction 95093) [order 2]
          state BUTTON_DOWN
            state Button_DOWN_1
              en:
              BUTTON_DOWN(2)=true;
              BUT_TEMP=1;
              LPD1=true;
              PUSHED=true;
              UPDATE=false;
              IN_LL=false; ET_LL=0;
            state First_but_1
              en:
              BUT_1=BUT_TEMP;
              FIRST_BUT=false;
            state Button_DOWN_2
              en:
              BUTTON_DOWN(3)=true;
              BUT_TEMP=2;
              LPD2=true;
              PUSHED=true;
              UPDATE=false;
              IN_LL=false; ET_LL=0;
            state First_but_2
              en:
              BUT_1=BUT_TEMP;
              FIRST_BUT=false;
            state Button_DOWN_3
              en:
              BUTTON_DOWN(4)=true;
              BUT_TEMP=3;
              LPD3=true;
              PUSHED=true;
              UPDATE=false;
              IN_LL=false; ET_LL=0;
            state First_but_3
              en:
              BUT_1=BUT_TEMP;
              FIRST_BUT=false;
            (default) -> (junction 95107)
            (junction 95107) -> Emergency.Doors.Opening3.Button_detection1.BUTTON_DOWN.Button_DOWN_1 [order 1] : [PD1]
            Emergency.Doors.Opening3.Button_detection1.BUTTON_DOWN.Button_DOWN_1 -> (junction 95108)
            (junction 95108) -> Emergency.Doors.Opening3.Button_detection1.BUTTON_DOWN.First_but_1 [order 1] : [FIRST_BUT && not(RPC1)]
            Emergency.Doors.Opening3.Button_detection1.BUTTON_DOWN.First_but_1 -> (junction 95109)
            (junction 95107) -> (junction 95110) [order 2]
            (junction 95108) -> (junction 95111) [order 2]
            (junction 95109) -> (junction 95112)
            (junction 95111) -> (junction 95110)
            (junction 95112) -> (junction 95111)
            (junction 95110) -> (junction 95113)
            (junction 95113) -> Emergency.Doors.Opening3.Button_detection1.BUTTON_DOWN.Button_DOWN_2 [order 1] : [PD2]
            Emergency.Doors.Opening3.Button_detection1.BUTTON_DOWN.Button_DOWN_2 -> (junction 95114)
            (junction 95114) -> Emergency.Doors.Opening3.Button_detection1.BUTTON_DOWN.First_but_2 [order 1] : [FIRST_BUT && not(RPC2)]
            Emergency.Doors.Opening3.Button_detection1.BUTTON_DOWN.First_but_2 -> (junction 95115)
            (junction 95113) -> (junction 95116) [order 2]
            (junction 95114) -> (junction 95117) [order 2]
            (junction 95115) -> (junction 95118)
            (junction 95117) -> (junction 95116)
            (junction 95118) -> (junction 95117)
            (junction 95116) -> (junction 95119)
            (junction 95119) -> Emergency.Doors.Opening3.Button_detection1.BUTTON_DOWN.Button_DOWN_3 [order 1] : [PD3]
            Emergency.Doors.Opening3.Button_detection1.BUTTON_DOWN.Button_DOWN_3 -> (junction 95120)
            (junction 95120) -> Emergency.Doors.Opening3.Button_detection1.BUTTON_DOWN.First_but_3 [order 1] : [FIRST_BUT && not(RPC3)]
            Emergency.Doors.Opening3.Button_detection1.BUTTON_DOWN.First_but_3 -> (junction 95121)
            (junction 95119) -> (junction 95122) [order 2]
            (junction 95120) -> (junction 95123) [order 2]
            (junction 95121) -> (junction 95124)
            (junction 95123) -> (junction 95122)
            (junction 95124) -> (junction 95123)
          state BUTTON_CAR
            state Button_CAR_0
              en:
              BUTTON_CAR(1)=true;
              BUT_TEMP=0;
              LPC0=true;
              PUSHED=true;
              UPDATE=false;
              IN_LL=false; ET_LL=0;
            state First_but_0
              en:
              BUT_1=BUT_TEMP;
              FIRST_BUT=false;
            state Button_CAR_1
              en:
              BUTTON_CAR(2)=true;
              BUT_TEMP=1;
              LPC1=true;
              PUSHED=true;
              UPDATE=false;
              IN_LL=false; ET_LL=0;
            state First_but_1
              en:
              BUT_1=BUT_TEMP;
              FIRST_BUT=false;
            state Button_CAR_2
              en:
              BUTTON_CAR(3)=true;
              BUT_TEMP=2;
              LPC2=true;
              PUSHED=true;
              UPDATE=false;
              IN_LL=false; ET_LL=0;
            state First_but_2
              en:
              BUT_1=BUT_TEMP;
              FIRST_BUT=false;
            state Button_CAR_3
              en:
              BUTTON_CAR(4)=true;
              BUT_TEMP=3;
              LPC3=true;
              PUSHED=true;
              UPDATE=false;
              IN_LL=false; ET_LL=0;
            state First_but_3
              en:
              BUT_1=BUT_TEMP;
              FIRST_BUT=false;
            (default) -> (junction 95162)
            (junction 95162) -> Emergency.Doors.Opening3.Button_detection1.BUTTON_CAR.Button_CAR_0 [order 1] : [P0]
            Emergency.Doors.Opening3.Button_detection1.BUTTON_CAR.Button_CAR_0 -> (junction 95163)
            (junction 95163) -> Emergency.Doors.Opening3.Button_detection1.BUTTON_CAR.First_but_0 [order 1] : [FIRST_BUT && not(RPC0)]
            Emergency.Doors.Opening3.Button_detection1.BUTTON_CAR.First_but_0 -> (junction 95164)
            (junction 95162) -> (junction 95165) [order 2]
            (junction 95163) -> (junction 95166) [order 2]
            (junction 95164) -> (junction 95167)
            (junction 95166) -> (junction 95165)
            (junction 95167) -> (junction 95166)
            (junction 95165) -> (junction 95170)
            Emergency.Doors.Opening3.Button_detection1.BUTTON_CAR.Button_CAR_1 -> (junction 95168)
            (junction 95168) -> Emergency.Doors.Opening3.Button_detection1.BUTTON_CAR.First_but_1 [order 1] : [FIRST_BUT && not(RPC1)]
            Emergency.Doors.Opening3.Button_detection1.BUTTON_CAR.First_but_1 -> (junction 95169)
            (junction 95168) -> (junction 95172) [order 2]
            (junction 95169) -> (junction 95173)
            (junction 95170) -> Emergency.Doors.Opening3.Button_detection1.BUTTON_CAR.Button_CAR_1 [order 1] : [P1]
            (junction 95170) -> (junction 95171) [order 2]
            (junction 95172) -> (junction 95171)
            (junction 95173) -> (junction 95172)
            (junction 95171) -> (junction 95174)
            (junction 95174) -> Emergency.Doors.Opening3.Button_detection1.BUTTON_CAR.Button_CAR_2 [order 1] : [P2]
            Emergency.Doors.Opening3.Button_detection1.BUTTON_CAR.Button_CAR_2 -> (junction 95175)
            (junction 95175) -> Emergency.Doors.Opening3.Button_detection1.BUTTON_CAR.First_but_2 [order 1] : [FIRST_BUT && not(RPC2)]
            Emergency.Doors.Opening3.Button_detection1.BUTTON_CAR.First_but_2 -> (junction 95176)
            (junction 95174) -> (junction 95177) [order 2]
            (junction 95175) -> (junction 95178) [order 2]
            (junction 95176) -> (junction 95179)
            (junction 95178) -> (junction 95177)
            (junction 95179) -> (junction 95178)
            (junction 95177) -> (junction 95180)
            (junction 95180) -> Emergency.Doors.Opening3.Button_detection1.BUTTON_CAR.Button_CAR_3 [order 1] : [P3]
            Emergency.Doors.Opening3.Button_detection1.BUTTON_CAR.Button_CAR_3 -> (junction 95181)
            (junction 95181) -> Emergency.Doors.Opening3.Button_detection1.BUTTON_CAR.First_but_3 [order 1] : [FIRST_BUT && not(RPC3)]
            Emergency.Doors.Opening3.Button_detection1.BUTTON_CAR.First_but_3 -> (junction 95182)
            (junction 95180) -> (junction 95183) [order 2]
            (junction 95181) -> (junction 95184) [order 2]
            (junction 95182) -> (junction 95185)
            (junction 95184) -> (junction 95183)
            (junction 95185) -> (junction 95184)
          state BUTTON_UP
            state Button_UP_0
              en:
              BUTTON_UP(1)=true;
              BUT_TEMP=0;
              LPS0=true;
              PUSHED=true;
              UPDATE=false;
              IN_LL=false; ET_LL=0;
            state First_but_0
              en:
              BUT_1=BUT_TEMP;
              FIRST_BUT=false;
            state Button_UP_1
              en:
              BUTTON_UP(2)=true;
              BUT_TEMP=1;
              LPS1=true;
              PUSHED=true;
              UPDATE=false;
              IN_LL=false; ET_LL=0;
            state First_but_1
              en:
              BUT_1=BUT_TEMP;
              FIRST_BUT=false;
            state Button_UP_2
              en:
              BUTTON_UP(3)=true;
              BUT_TEMP=2;
              LPS2=true;
              PUSHED=true;
              UPDATE=false;
              IN_LL=false; ET_LL=0;
            state First_but_2
              en:
              BUT_1=BUT_TEMP;
              FIRST_BUT=false;
            (junction 95235) -> Emergency.Doors.Opening3.Button_detection1.BUTTON_UP.Button_UP_0 [order 1] : [PS0]
            Emergency.Doors.Opening3.Button_detection1.BUTTON_UP.Button_UP_0 -> (junction 95236)
            (junction 95236) -> Emergency.Doors.Opening3.Button_detection1.BUTTON_UP.First_but_0 [order 1] : [FIRST_BUT && not(RPC0)]
            Emergency.Doors.Opening3.Button_detection1.BUTTON_UP.First_but_0 -> (junction 95237)
            (default) -> (junction 95235)
            (junction 95235) -> (junction 95240) [order 2]
            (junction 95236) -> (junction 95238) [order 2]
            (junction 95237) -> (junction 95239)
            (junction 95239) -> (junction 95238)
            (junction 95238) -> (junction 95240)
            (junction 95240) -> (junction 95241)
            (junction 95241) -> Emergency.Doors.Opening3.Button_detection1.BUTTON_UP.Button_UP_1 [order 1] : [PS1]
            Emergency.Doors.Opening3.Button_detection1.BUTTON_UP.Button_UP_1 -> (junction 95242)
            (junction 95242) -> Emergency.Doors.Opening3.Button_detection1.BUTTON_UP.First_but_1 [order 1] : [FIRST_BUT && not(RPC1)]
            Emergency.Doors.Opening3.Button_detection1.BUTTON_UP.First_but_1 -> (junction 95243)
            (junction 95241) -> (junction 95244) [order 2]
            (junction 95242) -> (junction 95245) [order 2]
            (junction 95243) -> (junction 95246)
            (junction 95245) -> (junction 95244)
            (junction 95246) -> (junction 95245)
            (junction 95244) -> (junction 95248)
            Emergency.Doors.Opening3.Button_detection1.BUTTON_UP.First_but_2 -> (junction 95247)
            (junction 95247) -> (junction 95252)
            (junction 95248) -> Emergency.Doors.Opening3.Button_detection1.BUTTON_UP.Button_UP_2 [order 1] : [PS2]
            Emergency.Doors.Opening3.Button_detection1.BUTTON_UP.Button_UP_2 -> (junction 95249)
            (junction 95249) -> Emergency.Doors.Opening3.Button_detection1.BUTTON_UP.First_but_2 [order 1] : [FIRST_BUT && not(RPC2)]
            (junction 95248) -> (junction 95250) [order 2]
            (junction 95249) -> (junction 95251) [order 2]
            (junction 95251) -> (junction 95250)
            (junction 95252) -> (junction 95251)
          state Max_Min_assignment
            state Min_but
              en:
              BUTTON=MIN_BUT;
            state Max_but
              en:
              BUTTON=MAX_BUT;
            state First_but
              en:
              BUTTON=BUT_1;
            state Max_but1
              en:
              MAX_BUT=2;
            state Max_but2
              en:
              MAX_BUT=1;
            state Max_but3
              en:
              MAX_BUT=0;
            state Min_but1
              en:
              MIN_BUT=1;
            state Min_but2
              en:
              MIN_BUT=2;
            state Min_but3
              en:
              MIN_BUT=3;
            state MAX
              en:
              MAX_BUT=BUT_TEMP;
            state MIN
              en:
              MIN_BUT=BUT_TEMP;
            state Updating_button_0
              en:
              BUTTON=MAX_BUT;
            state Updating_button_1
              en:
              BUTTON=MIN_BUT;
            (junction 95290) -> Emergency.Doors.Opening3.Button_detection1.Max_Min_assignment.Min_but [order 1] : [(MAX_BUT-FLOOR)>(FLOOR-MIN_BUT)]
            Emergency.Doors.Opening3.Button_detection1.Max_Min_assignment.Min_but -> (junction 95291)
            (junction 95292) -> (junction 95290) [order 1] : [not(FLAG_STOP) && MOTION==2 && FLAG==3]
            (default) -> (junction 95292)
            (junction 95290) -> (junction 95293) [order 2]
            (junction 95291) -> (junction 95294)
            (junction 95292) -> (junction 95295) [order 2]
            (junction 95293) -> Emergency.Doors.Opening3.Button_detection1.Max_Min_assignment.Max_but [order 1] : [(MAX_BUT-FLOOR)<(FLOOR-MIN_BUT)]
            Emergency.Doors.Opening3.Button_detection1.Max_Min_assignment.Max_but -> (junction 95294)
            (junction 95293) -> Emergency.Doors.Opening3.Button_detection1.Max_Min_assignment.First_but [order 2]
            (junction 95294) -> (junction 95297)
            Emergency.Doors.Opening3.Button_detection1.Max_Min_assignment.First_but -> (junction 95296)
            (junction 95296) -> (junction 95295)
            (junction 95297) -> (junction 95296)
            (junction 95295) -> (junction 95298)
            (junction 95299) -> (junction 95300) [order 1] : [MOTION==0]
                | {MOTION=1;
                | UPDATE=true;}
            (junction 95300) -> Emergency.Doors.Opening3.Button_detection1.Max_Min_assignment.Max_but1 [order 1] : [BUTTON_UP(2)]
            Emergency.Doors.Opening3.Button_detection1.Max_Min_assignment.Max_but1 -> (junction 95301)
            (junction 95298) -> (junction 95299) [order 1] : [BUTTON==FLOOR && EXTEND]
                | {EXTEND=false;}
            (junction 95298) -> (junction 95312) [order 2]
            (junction 95299) -> (junction 95304) [order 2]
            (junction 95300) -> (junction 95302) [order 2]
            (junction 95301) -> (junction 95303)
            (junction 95302) -> Emergency.Doors.Opening3.Button_detection1.Max_Min_assignment.Max_but2 [order 1] : [BUTTON_UP(1)]
            Emergency.Doors.Opening3.Button_detection1.Max_Min_assignment.Max_but2 -> (junction 95303)
            (junction 95302) -> Emergency.Doors.Opening3.Button_detection1.Max_Min_assignment.Max_but3 [order 2]
            (junction 95303) -> (junction 95306)
            Emergency.Doors.Opening3.Button_detection1.Max_Min_assignment.Max_but3 -> (junction 95305)
            (junction 95305) -> (junction 95304)
            (junction 95306) -> (junction 95305)
            (junction 95304) -> (junction 95307)
            (junction 95307) -> (junction 95308) [order 1] : [MOTION==1]
                | {MOTION=0;
                | UPDATE=true;}
            (junction 95308) -> Emergency.Doors.Opening3.Button_detection1.Max_Min_assignment.Min_but1 [order 1] : [BUTTON_DOWN(1)]
            Emergency.Doors.Opening3.Button_detection1.Max_Min_assignment.Min_but1 -> (junction 95309)
            (junction 95307) -> (junction 95313) [order 2]
            (junction 95308) -> (junction 95310) [order 2]
            (junction 95309) -> (junction 95311)
            (junction 95310) -> Emergency.Doors.Opening3.Button_detection1.Max_Min_assignment.Min_but2 [order 1] : [BUTTON_DOWN(2)]
            Emergency.Doors.Opening3.Button_detection1.Max_Min_assignment.Min_but2 -> (junction 95311)
            (junction 95310) -> Emergency.Doors.Opening3.Button_detection1.Max_Min_assignment.Min_but3 [order 2]
            (junction 95311) -> (junction 95315)
            Emergency.Doors.Opening3.Button_detection1.Max_Min_assignment.Min_but3 -> (junction 95314)
            (junction 95313) -> (junction 95312)
            (junction 95314) -> (junction 95313)
            (junction 95315) -> (junction 95314)
            (junction 95312) -> (junction 95317)
            Emergency.Doors.Opening3.Button_detection1.Max_Min_assignment.MAX -> (junction 95316)
            (junction 95317) -> (junction 95318) [order 1] : [PUSHED]
            (junction 95318) -> (junction 95319) [order 1] : [not(BUT_TEMP==FLOOR) || not(MOTION==2)]
            (junction 95319) -> Emergency.Doors.Opening3.Button_detection1.Max_Min_assignment.MAX [order 1] : [MAX_BUT<BUT_TEMP && not(UPDATE)]
            (junction 95316) -> (junction 95321)
            (junction 95317) -> (junction 95331) [order 2]
            (junction 95318) -> (junction 95324) [order 2]
            (junction 95319) -> (junction 95320) [order 2]
            (junction 95321) -> (junction 95320)
            (junction 95320) -> (junction 95322)
            (junction 95322) -> Emergency.Doors.Opening3.Button_detection1.Max_Min_assignment.MIN [order 1] : [MIN_BUT>BUT_TEMP && not(UPDATE)]
            Emergency.Doors.Opening3.Button_detection1.Max_Min_assignment.MIN -> (junction 95323)
            (junction 95322) -> (junction 95325) [order 2]
            (junction 95323) -> (junction 95326)
            (junction 95325) -> (junction 95324)
            (junction 95326) -> (junction 95325)
            (junction 95324) -> (junction 95327)
            (junction 95327) -> Emergency.Doors.Opening3.Button_detection1.Max_Min_assignment.Updating_button_0 [order 1] : [MOTION==0]
            Emergency.Doors.Opening3.Button_detection1.Max_Min_assignment.Updating_button_0 -> (junction 95328)
            (junction 95327) -> (junction 95329) [order 2]
            (junction 95328) -> (junction 95330)
            (junction 95329) -> Emergency.Doors.Opening3.Button_detection1.Max_Min_assignment.Updating_button_1 [order 1] : [MOTION==1]
            Emergency.Doors.Opening3.Button_detection1.Max_Min_assignment.Updating_button_1 -> (junction 95330)
            (junction 95329) -> (junction 95332) [order 2]
            (junction 95330) -> (junction 95333)
            (junction 95332) -> (junction 95331)
            (junction 95333) -> (junction 95332)
          state GoTo_PositionControl
            en:
            BUTTON=BUT_TEMP;
            FLAG=2;
          state Emergency
            en:
            FLAG_EMG=true;
            FLAG=4;
          state Timer_EME
            state Set_tmr
              en:
              Q_EME=true;
            state Counting
              en:
              ET_EME= ET_EME + 1;
              Q_EME=false;
            state Set
              en:
              IN_EME=true;
              PT_EME=3;
            (junction 95423) -> Emergency.Doors.Opening3.Button_detection1.Timer_EME.Set_tmr [order 1] : [ET_EME==PT_EME]
            Emergency.Doors.Opening3.Button_detection1.Timer_EME.Set_tmr -> (junction 95424)
            Emergency.Doors.Opening3.Button_detection1.Timer_EME.Counting -> (junction 95423)
            (junction 95423) -> (junction 95424) [order 2]
            (default) -> Emergency.Doors.Opening3.Button_detection1.Timer_EME.Set
            Emergency.Doors.Opening3.Button_detection1.Timer_EME.Set -> (junction 95425)
            (junction 95425) -> Emergency.Doors.Opening3.Button_detection1.Timer_EME.Counting [order 1] : [ET_EME<PT_EME]
            (junction 95425) -> (junction 95424) [order 2]
          state Not_Emergency
            en:
            IN_EME=false;
            ET_EME=0;
          state SwitchingOFF_LEDs
            en:
            LPD3=false;
            LPD2=false;
            LPS2=false;
            LPD1=false;
            LPS1=false;
            LPS0=false;
          (default) -> (junction 95024)
          (junction 95024) -> (junction 95025) [order 1] : [FLAG==1 && not(PUSHED)]
              | {BUTTON=FLOOR;
              | BUT_TEMP=BUTTON;
              | BUT_1=FLOOR;}
          (junction 95025) -> Emergency.Doors.Opening3.Button_detection1.Timer_LL [order 1] : [not(FLAG_STOP)]
          Emergency.Doors.Opening3.Button_detection1.Save_energy -> (junction 95026)
          Emergency.Doors.Opening3.Button_detection1.Timer_LL -> Emergency.Doors.Opening3.Button_detection1.Save_energy
          (junction 95025) -> (junction 95028) [order 2]
          (junction 95024) -> (junction 95027) [order 2]
          (junction 95026) -> (junction 95029)
          (junction 95028) -> (junction 95027)
          (junction 95029) -> (junction 95028)
          (junction 95027) -> Emergency.Doors.Opening3.Button_detection1.BUTTON_CAR
          Emergency.Doors.Opening3.Button_detection1.BUTTON_UP -> Emergency.Doors.Opening3.Button_detection1.BUTTON_DOWN
          Emergency.Doors.Opening3.Button_detection1.BUTTON_DOWN -> Emergency.Doors.Opening3.Button_detection1.Max_Min_assignment
          Emergency.Doors.Opening3.Button_detection1.Max_Min_assignment -> (junction 95030)
          Emergency.Doors.Opening3.Button_detection1.BUTTON_CAR -> Emergency.Doors.Opening3.Button_detection1.BUTTON_UP
          (junction 95030) -> (junction 95032)
          (junction 95032) -> (junction 95031)
          (junction 95031) -> (junction 95034)
          Emergency.Doors.Opening3.Button_detection1.GoTo_PositionControl -> (junction 95033)
          (junction 95034) -> (junction 95035) [order 1] : [FLAG==1]
          (junction 95035) -> Emergency.Doors.Opening3.Button_detection1.GoTo_PositionControl [order 1] : [PUSHED]
          (junction 95033) -> (junction 95037)
          (junction 95034) -> (junction 95045) [order 2]
          (junction 95035) -> (junction 95036) [order 2]
          (junction 95037) -> (junction 95036)
          (junction 95036) -> (junction 95039)
          Emergency.Doors.Opening3.Button_detection1.Emergency -> (junction 95038)
          (junction 95039) -> Emergency.Doors.Opening3.Button_detection1.Timer_EME [order 1] : [STOP]
              | {IN_LL=false; ET_LL=0;FLAG=1;}
          Emergency.Doors.Opening3.Button_detection1.Timer_EME -> (junction 95040)
          (junction 95040) -> Emergency.Doors.Opening3.Button_detection1.Emergency [order 1] : [Q_EME]
          (junction 95038) -> (junction 95042)
          (junction 95039) -> Emergency.Doors.Opening3.Button_detection1.Not_Emergency [order 2]
          (junction 95040) -> (junction 95041) [order 2]
          (junction 95042) -> (junction 95041)
          (junction 95041) -> (junction 95044)
          Emergency.Doors.Opening3.Button_detection1.Not_Emergency -> (junction 95044)
          Emergency.Doors.Opening3.Button_detection1.SwitchingOFF_LEDs -> (junction 95043)
          (junction 95044) -> Emergency.Doors.Opening3.Button_detection1.SwitchingOFF_LEDs [order 1] : [FLAG_STOP && FLAG==2]
          (junction 95043) -> (junction 95047)
          (junction 95044) -> (junction 95046) [order 2]
          (junction 95046) -> (junction 95045)
          (junction 95047) -> (junction 95046)
        state Opening1
          en:AP3=true;
        state Reset
          state Reset_0
            en:
            LPS0=false;
            BUTTON_CAR(1)=false;
            BUTTON_UP(1)=false;
          state Reset_1
            en:
            LPS1=false;
            LPD1=false;
            BUTTON_CAR(2)=false;
            BUTTON_UP(2)=false;
            BUTTON_DOWN(2)=false;
          state Reset_2
            en:
            LPS2=false;
            LPD2=false;
            BUTTON_CAR(3)=false;
            BUTTON_UP(3)=false;
            BUTTON_DOWN(3)=false;
          state Reset_3
            en:
            LPD3=false;
            BUTTON_CAR(4)=false;
            BUTTON_DOWN(4)=false;
          (default) -> (junction 95441)
          (junction 95441) -> Emergency.Doors.Opening3.Reset.Reset_0 [order 1] : [FLOOR==0]
          Emergency.Doors.Opening3.Reset.Reset_0 -> (junction 95442)
          (junction 95441) -> (junction 95443) [order 2]
          (junction 95442) -> (junction 95444)
          (junction 95443) -> Emergency.Doors.Opening3.Reset.Reset_1 [order 1] : [FLOOR==1]
          Emergency.Doors.Opening3.Reset.Reset_1 -> (junction 95444)
          (junction 95443) -> (junction 95445) [order 2]
          (junction 95444) -> (junction 95446)
          (junction 95445) -> Emergency.Doors.Opening3.Reset.Reset_2 [order 1] : [FLOOR==2]
          Emergency.Doors.Opening3.Reset.Reset_2 -> (junction 95446)
          (junction 95445) -> (junction 95447) [order 2]
          (junction 95446) -> (junction 95448)
          (junction 95447) -> Emergency.Doors.Opening3.Reset.Reset_3 [order 1] : [FLOOR==3]
          Emergency.Doors.Opening3.Reset.Reset_3 -> (junction 95448)
          (junction 95447) -> (junction 95449) [order 2]
          (junction 95448) -> (junction 95450)
          (junction 95450) -> (junction 95449)
        state Stop_Opening1
          en: AP3=false;
          FLAG_OD=true;
          IN_cl=false;
          ET_cl=0;
        (junction 94438) -> (junction 94439)
        (junction 94439) -> (junction 94440) [order 1] : [not(OBS) ]
        (junction 94442) -> Emergency.Doors.Opening3.Opening [order 1] : [not(PA3)]
        (junction 94440) -> (junction 94441) [order 2]
        (junction 94441) -> Emergency.Doors.Opening3.Timer_open
        Emergency.Doors.Opening3.Timer_open -> (junction 94442)
        (default) -> Emergency.Doors.Opening3.People_IN
        (junction 94439) -> (junction 94443) [order 2]
        (junction 94440) -> Emergency.Doors.Opening3.Button_detection [order 1] : [not(FLAG==4)]
        (junction 94445) -> (junction 94441)
        (junction 94447) -> (junction 94438)
        (junction 94442) -> Emergency.Doors.Opening3.Stop_Opening [order 2]
        Emergency.Doors.Opening3.People_IN -> Emergency.Doors.Opening3.People_OUT
        Emergency.Doors.Opening3.Opening -> (junction 94452)
        (junction 94443) -> (junction 94444) [order 2]
        (junction 94443) -> Emergency.Doors.Opening3.Button_detection1 [order 1] : [not(FLAG==4)]
        (junction 94444) -> (junction 94449)
        Emergency.Doors.Opening3.Button_detection -> (junction 94445)
        Emergency.Doors.Opening3.People_OUT -> (junction 94446)
        Emergency.Doors.Opening3.Button_detection1 -> (junction 94448)
        (junction 94449) -> (junction 94448)
        (junction 94446) -> (junction 94447) [order 2]
        (junction 94446) -> Emergency.Doors.Opening3.Reset [order 1] : [not(FLAG==4)]
        (junction 94448) -> (junction 94450)
        (junction 94456) -> (junction 94447)
        Emergency.Doors.Opening3.Stop_Opening -> (junction 94451)
        (junction 94450) -> Emergency.Doors.Opening3.Opening1 [order 1] : [not(PA3)]
        (junction 94450) -> Emergency.Doors.Opening3.Stop_Opening1 [order 2]
        (junction 94452) -> (junction 94451)
        (junction 94451) -> (junction 94454)
        Emergency.Doors.Opening3.Opening1 -> (junction 94453)
        Emergency.Doors.Opening3.Reset -> (junction 94455)
        Emergency.Doors.Opening3.Stop_Opening1 -> (junction 94453)
        (junction 94453) -> (junction 94454)
        (junction 94455) -> (junction 94456)
      state Closing0
        state Reset
          state Reset_0
            en:
            LPS0=false;
            BUTTON_CAR(1)=false;
            BUTTON_UP(1)=false;
          state Reset_1
            en:
            LPS1=false;
            LPD1=false;
            BUTTON_CAR(2)=false;
            BUTTON_UP(2)=false;
            BUTTON_DOWN(2)=false;
          state Reset_2
            en:
            LPS2=false;
            LPD2=false;
            BUTTON_CAR(3)=false;
            BUTTON_UP(3)=false;
            BUTTON_DOWN(3)=false;
          state Reset_3
            en:
            LPD3=false;
            BUTTON_CAR(4)=false;
            BUTTON_DOWN(4)=false;
          (default) -> (junction 78931)
          (junction 78931) -> Emergency.Doors.Closing0.Reset.Reset_0 [order 1] : [FLOOR==0]
          Emergency.Doors.Closing0.Reset.Reset_0 -> (junction 78932)
          (junction 78931) -> (junction 78933) [order 2]
          (junction 78932) -> (junction 78934)
          (junction 78933) -> Emergency.Doors.Closing0.Reset.Reset_1 [order 1] : [FLOOR==1]
          Emergency.Doors.Closing0.Reset.Reset_1 -> (junction 78934)
          (junction 78933) -> (junction 78935) [order 2]
          (junction 78934) -> (junction 78936)
          (junction 78935) -> Emergency.Doors.Closing0.Reset.Reset_2 [order 1] : [FLOOR==2]
          Emergency.Doors.Closing0.Reset.Reset_2 -> (junction 78936)
          (junction 78935) -> (junction 78937) [order 2]
          (junction 78936) -> (junction 78938)
          (junction 78937) -> Emergency.Doors.Closing0.Reset.Reset_3 [order 1] : [FLOOR==3]
          Emergency.Doors.Closing0.Reset.Reset_3 -> (junction 78938)
          (junction 78937) -> (junction 78939) [order 2]
          (junction 78938) -> (junction 78940)
          (junction 78940) -> (junction 78939)
        state Timer_close
          state Set_tmr
            en: Q_cl=true;
          state Set
            en:PT_cl=5;
            IN_cl=true;
          state Counting
            en:ET_cl = ET_cl + 1;
            Q_cl=false;
          (junction 78964) -> Emergency.Doors.Closing0.Timer_close.Set_tmr [order 1] : [ET_cl==PT_cl]
          Emergency.Doors.Closing0.Timer_close.Set_tmr -> (junction 78965)
          (default) -> Emergency.Doors.Closing0.Timer_close.Set
          Emergency.Doors.Closing0.Timer_close.Counting -> (junction 78964)
          (junction 78964) -> (junction 78965) [order 2]
          Emergency.Doors.Closing0.Timer_close.Set -> (junction 78966)
          (junction 78966) -> Emergency.Doors.Closing0.Timer_close.Counting [order 1] : [ET_cl<PT_cl]
          (junction 78966) -> (junction 78965) [order 2]
        state Closing
          en: CP0=Q_cl;
        state Button_detection
          state Save_energy
            en:
            LL=not(Q_LL);
          state Timer_LL
            state Set_tmr
              en:
              Q_LL=true;
            state Counting
              en:
              ET_LL= ET_LL + 1;
              Q_LL=false;
            state Set
              en:
              IN_LL=true;
              PT_LL=10;
            (junction 79048) -> Emergency.Doors.Closing0.Button_detection.Timer_LL.Set_tmr [order 1] : [ET_LL==PT_LL]
            Emergency.Doors.Closing0.Button_detection.Timer_LL.Set_tmr -> (junction 79049)
            Emergency.Doors.Closing0.Button_detection.Timer_LL.Counting -> (junction 79048)
            (junction 79048) -> (junction 79049) [order 2]
            (default) -> Emergency.Doors.Closing0.Button_detection.Timer_LL.Set
            Emergency.Doors.Closing0.Button_detection.Timer_LL.Set -> (junction 79050)
            (junction 79050) -> Emergency.Doors.Closing0.Button_detection.Timer_LL.Counting [order 1] : [ET_LL<PT_LL]
            (junction 79050) -> (junction 79049) [order 2]
          state BUTTON_DOWN
            state Button_DOWN_1
              en:
              BUTTON_DOWN(2)=true;
              BUT_TEMP=1;
              LPD1=true;
              PUSHED=true;
              UPDATE=false;
              IN_LL=false; ET_LL=0;
            state First_but_1
              en:
              BUT_1=BUT_TEMP;
              FIRST_BUT=false;
            state Button_DOWN_2
              en:
              BUTTON_DOWN(3)=true;
              BUT_TEMP=2;
              LPD2=true;
              PUSHED=true;
              UPDATE=false;
              IN_LL=false; ET_LL=0;
            state First_but_2
              en:
              BUT_1=BUT_TEMP;
              FIRST_BUT=false;
            state Button_DOWN_3
              en:
              BUTTON_DOWN(4)=true;
              BUT_TEMP=3;
              LPD3=true;
              PUSHED=true;
              UPDATE=false;
              IN_LL=false; ET_LL=0;
            state First_but_3
              en:
              BUT_1=BUT_TEMP;
              FIRST_BUT=false;
            (default) -> (junction 79063)
            (junction 79063) -> Emergency.Doors.Closing0.Button_detection.BUTTON_DOWN.Button_DOWN_1 [order 1] : [PD1]
            Emergency.Doors.Closing0.Button_detection.BUTTON_DOWN.Button_DOWN_1 -> (junction 79064)
            (junction 79064) -> Emergency.Doors.Closing0.Button_detection.BUTTON_DOWN.First_but_1 [order 1] : [FIRST_BUT && not(RPC1)]
            Emergency.Doors.Closing0.Button_detection.BUTTON_DOWN.First_but_1 -> (junction 79065)
            (junction 79063) -> (junction 79066) [order 2]
            (junction 79064) -> (junction 79067) [order 2]
            (junction 79065) -> (junction 79068)
            (junction 79067) -> (junction 79066)
            (junction 79068) -> (junction 79067)
            (junction 79066) -> (junction 79069)
            (junction 79069) -> Emergency.Doors.Closing0.Button_detection.BUTTON_DOWN.Button_DOWN_2 [order 1] : [PD2]
            Emergency.Doors.Closing0.Button_detection.BUTTON_DOWN.Button_DOWN_2 -> (junction 79070)
            (junction 79070) -> Emergency.Doors.Closing0.Button_detection.BUTTON_DOWN.First_but_2 [order 1] : [FIRST_BUT && not(RPC2)]
            Emergency.Doors.Closing0.Button_detection.BUTTON_DOWN.First_but_2 -> (junction 79071)
            (junction 79069) -> (junction 79072) [order 2]
            (junction 79070) -> (junction 79073) [order 2]
            (junction 79071) -> (junction 79074)
            (junction 79073) -> (junction 79072)
            (junction 79074) -> (junction 79073)
            (junction 79072) -> (junction 79075)
            (junction 79075) -> Emergency.Doors.Closing0.Button_detection.BUTTON_DOWN.Button_DOWN_3 [order 1] : [PD3]
            Emergency.Doors.Closing0.Button_detection.BUTTON_DOWN.Button_DOWN_3 -> (junction 79076)
            (junction 79076) -> Emergency.Doors.Closing0.Button_detection.BUTTON_DOWN.First_but_3 [order 1] : [FIRST_BUT && not(RPC3)]
            Emergency.Doors.Closing0.Button_detection.BUTTON_DOWN.First_but_3 -> (junction 79077)
            (junction 79075) -> (junction 79078) [order 2]
            (junction 79076) -> (junction 79079) [order 2]
            (junction 79077) -> (junction 79080)
            (junction 79079) -> (junction 79078)
            (junction 79080) -> (junction 79079)
          state BUTTON_CAR
            state Button_CAR_0
              en:
              BUTTON_CAR(1)=true;
              BUT_TEMP=0;
              LPC0=true;
              PUSHED=true;
              UPDATE=false;
              IN_LL=false; ET_LL=0;
            state First_but_0
              en:
              BUT_1=BUT_TEMP;
              FIRST_BUT=false;
            state Button_CAR_1
              en:
              BUTTON_CAR(2)=true;
              BUT_TEMP=1;
              LPC1=true;
              PUSHED=true;
              UPDATE=false;
              IN_LL=false; ET_LL=0;
            state First_but_1
              en:
              BUT_1=BUT_TEMP;
              FIRST_BUT=false;
            state Button_CAR_2
              en:
              BUTTON_CAR(3)=true;
              BUT_TEMP=2;
              LPC2=true;
              PUSHED=true;
              UPDATE=false;
              IN_LL=false; ET_LL=0;
            state First_but_2
              en:
              BUT_1=BUT_TEMP;
              FIRST_BUT=false;
            state Button_CAR_3
              en:
              BUTTON_CAR(4)=true;
              BUT_TEMP=3;
              LPC3=true;
              PUSHED=true;
              UPDATE=false;
              IN_LL=false; ET_LL=0;
            state First_but_3
              en:
              BUT_1=BUT_TEMP;
              FIRST_BUT=false;
            (default) -> (junction 79118)
            (junction 79118) -> Emergency.Doors.Closing0.Button_detection.BUTTON_CAR.Button_CAR_0 [order 1] : [P0]
            Emergency.Doors.Closing0.Button_detection.BUTTON_CAR.Button_CAR_0 -> (junction 79119)
            (junction 79119) -> Emergency.Doors.Closing0.Button_detection.BUTTON_CAR.First_but_0 [order 1] : [FIRST_BUT && not(RPC0)]
            Emergency.Doors.Closing0.Button_detection.BUTTON_CAR.First_but_0 -> (junction 79120)
            (junction 79118) -> (junction 79121) [order 2]
            (junction 79119) -> (junction 79122) [order 2]
            (junction 79120) -> (junction 79123)
            (junction 79122) -> (junction 79121)
            (junction 79123) -> (junction 79122)
            (junction 79121) -> (junction 79126)
            Emergency.Doors.Closing0.Button_detection.BUTTON_CAR.Button_CAR_1 -> (junction 79124)
            (junction 79124) -> Emergency.Doors.Closing0.Button_detection.BUTTON_CAR.First_but_1 [order 1] : [FIRST_BUT && not(RPC1)]
            Emergency.Doors.Closing0.Button_detection.BUTTON_CAR.First_but_1 -> (junction 79125)
            (junction 79124) -> (junction 79128) [order 2]
            (junction 79125) -> (junction 79129)
            (junction 79126) -> Emergency.Doors.Closing0.Button_detection.BUTTON_CAR.Button_CAR_1 [order 1] : [P1]
            (junction 79126) -> (junction 79127) [order 2]
            (junction 79128) -> (junction 79127)
            (junction 79129) -> (junction 79128)
            (junction 79127) -> (junction 79130)
            (junction 79130) -> Emergency.Doors.Closing0.Button_detection.BUTTON_CAR.Button_CAR_2 [order 1] : [P2]
            Emergency.Doors.Closing0.Button_detection.BUTTON_CAR.Button_CAR_2 -> (junction 79131)
            (junction 79131) -> Emergency.Doors.Closing0.Button_detection.BUTTON_CAR.First_but_2 [order 1] : [FIRST_BUT && not(RPC2)]
            Emergency.Doors.Closing0.Button_detection.BUTTON_CAR.First_but_2 -> (junction 79132)
            (junction 79130) -> (junction 79133) [order 2]
            (junction 79131) -> (junction 79134) [order 2]
            (junction 79132) -> (junction 79135)
            (junction 79134) -> (junction 79133)
            (junction 79135) -> (junction 79134)
            (junction 79133) -> (junction 79136)
            (junction 79136) -> Emergency.Doors.Closing0.Button_detection.BUTTON_CAR.Button_CAR_3 [order 1] : [P3]
            Emergency.Doors.Closing0.Button_detection.BUTTON_CAR.Button_CAR_3 -> (junction 79137)
            (junction 79137) -> Emergency.Doors.Closing0.Button_detection.BUTTON_CAR.First_but_3 [order 1] : [FIRST_BUT && not(RPC3)]
            Emergency.Doors.Closing0.Button_detection.BUTTON_CAR.First_but_3 -> (junction 79138)
            (junction 79136) -> (junction 79139) [order 2]
            (junction 79137) -> (junction 79140) [order 2]
            (junction 79138) -> (junction 79141)
            (junction 79140) -> (junction 79139)
            (junction 79141) -> (junction 79140)
          state BUTTON_UP
            state Button_UP_0
              en:
              BUTTON_UP(1)=true;
              BUT_TEMP=0;
              LPS0=true;
              PUSHED=true;
              UPDATE=false;
              IN_LL=false; ET_LL=0;
            state First_but_0
              en:
              BUT_1=BUT_TEMP;
              FIRST_BUT=false;
            state Button_UP_1
              en:
              BUTTON_UP(2)=true;
              BUT_TEMP=1;
              LPS1=true;
              PUSHED=true;
              UPDATE=false;
              IN_LL=false; ET_LL=0;
            state First_but_1
              en:
              BUT_1=BUT_TEMP;
              FIRST_BUT=false;
            state Button_UP_2
              en:
              BUTTON_UP(3)=true;
              BUT_TEMP=2;
              LPS2=true;
              PUSHED=true;
              UPDATE=false;
              IN_LL=false; ET_LL=0;
            state First_but_2
              en:
              BUT_1=BUT_TEMP;
              FIRST_BUT=false;
            (junction 79191) -> Emergency.Doors.Closing0.Button_detection.BUTTON_UP.Button_UP_0 [order 1] : [PS0]
            Emergency.Doors.Closing0.Button_detection.BUTTON_UP.Button_UP_0 -> (junction 79192)
            (junction 79192) -> Emergency.Doors.Closing0.Button_detection.BUTTON_UP.First_but_0 [order 1] : [FIRST_BUT && not(RPC0)]
            Emergency.Doors.Closing0.Button_detection.BUTTON_UP.First_but_0 -> (junction 79193)
            (default) -> (junction 79191)
            (junction 79191) -> (junction 79196) [order 2]
            (junction 79192) -> (junction 79194) [order 2]
            (junction 79193) -> (junction 79195)
            (junction 79195) -> (junction 79194)
            (junction 79194) -> (junction 79196)
            (junction 79196) -> (junction 79197)
            (junction 79197) -> Emergency.Doors.Closing0.Button_detection.BUTTON_UP.Button_UP_1 [order 1] : [PS1]
            Emergency.Doors.Closing0.Button_detection.BUTTON_UP.Button_UP_1 -> (junction 79198)
            (junction 79198) -> Emergency.Doors.Closing0.Button_detection.BUTTON_UP.First_but_1 [order 1] : [FIRST_BUT && not(RPC1)]
            Emergency.Doors.Closing0.Button_detection.BUTTON_UP.First_but_1 -> (junction 79199)
            (junction 79197) -> (junction 79200) [order 2]
            (junction 79198) -> (junction 79201) [order 2]
            (junction 79199) -> (junction 79202)
            (junction 79201) -> (junction 79200)
            (junction 79202) -> (junction 79201)
            (junction 79200) -> (junction 79204)
            Emergency.Doors.Closing0.Button_detection.BUTTON_UP.First_but_2 -> (junction 79203)
            (junction 79203) -> (junction 79208)
            (junction 79204) -> Emergency.Doors.Closing0.Button_detection.BUTTON_UP.Button_UP_2 [order 1] : [PS2]
            Emergency.Doors.Closing0.Button_detection.BUTTON_UP.Button_UP_2 -> (junction 79205)
            (junction 79205) -> Emergency.Doors.Closing0.Button_detection.BUTTON_UP.First_but_2 [order 1] : [FIRST_BUT && not(RPC2)]
            (junction 79204) -> (junction 79206) [order 2]
            (junction 79205) -> (junction 79207) [order 2]
            (junction 79207) -> (junction 79206)
            (junction 79208) -> (junction 79207)
          state Max_Min_assignment
            state Min_but
              en:
              BUTTON=MIN_BUT;
            state Max_but
              en:
              BUTTON=MAX_BUT;
            state First_but
              en:
              BUTTON=BUT_1;
            state Max_but1
              en:
              MAX_BUT=2;
            state Max_but2
              en:
              MAX_BUT=1;
            state Max_but3
              en:
              MAX_BUT=0;
            state Min_but1
              en:
              MIN_BUT=1;
            state Min_but2
              en:
              MIN_BUT=2;
            state Min_but3
              en:
              MIN_BUT=3;
            state MAX
              en:
              MAX_BUT=BUT_TEMP;
            state MIN
              en:
              MIN_BUT=BUT_TEMP;
            state Updating_button_0
              en:
              BUTTON=MAX_BUT;
            state Updating_button_1
              en:
              BUTTON=MIN_BUT;
            (junction 79246) -> Emergency.Doors.Closing0.Button_detection.Max_Min_assignment.Min_but [order 1] : [(MAX_BUT-FLOOR)>(FLOOR-MIN_BUT)]
            Emergency.Doors.Closing0.Button_detection.Max_Min_assignment.Min_but -> (junction 79247)
            (junction 79248) -> (junction 79246) [order 1] : [not(FLAG_STOP) && MOTION==2 && FLAG==3]
            (default) -> (junction 79248)
            (junction 79246) -> (junction 79249) [order 2]
            (junction 79247) -> (junction 79250)
            (junction 79248) -> (junction 79251) [order 2]
            (junction 79249) -> Emergency.Doors.Closing0.Button_detection.Max_Min_assignment.Max_but [order 1] : [(MAX_BUT-FLOOR)<(FLOOR-MIN_BUT)]
            Emergency.Doors.Closing0.Button_detection.Max_Min_assignment.Max_but -> (junction 79250)
            (junction 79249) -> Emergency.Doors.Closing0.Button_detection.Max_Min_assignment.First_but [order 2]
            (junction 79250) -> (junction 79253)
            Emergency.Doors.Closing0.Button_detection.Max_Min_assignment.First_but -> (junction 79252)
            (junction 79252) -> (junction 79251)
            (junction 79253) -> (junction 79252)
            (junction 79251) -> (junction 79254)
            (junction 79255) -> (junction 79256) [order 1] : [MOTION==0]
                | {MOTION=1;
                | UPDATE=true;}
            (junction 79256) -> Emergency.Doors.Closing0.Button_detection.Max_Min_assignment.Max_but1 [order 1] : [BUTTON_UP(2)]
            Emergency.Doors.Closing0.Button_detection.Max_Min_assignment.Max_but1 -> (junction 79257)
            (junction 79254) -> (junction 79255) [order 1] : [BUTTON==FLOOR && EXTEND]
                | {EXTEND=false;}
            (junction 79254) -> (junction 79268) [order 2]
            (junction 79255) -> (junction 79260) [order 2]
            (junction 79256) -> (junction 79258) [order 2]
            (junction 79257) -> (junction 79259)
            (junction 79258) -> Emergency.Doors.Closing0.Button_detection.Max_Min_assignment.Max_but2 [order 1] : [BUTTON_UP(1)]
            Emergency.Doors.Closing0.Button_detection.Max_Min_assignment.Max_but2 -> (junction 79259)
            (junction 79258) -> Emergency.Doors.Closing0.Button_detection.Max_Min_assignment.Max_but3 [order 2]
            (junction 79259) -> (junction 79262)
            Emergency.Doors.Closing0.Button_detection.Max_Min_assignment.Max_but3 -> (junction 79261)
            (junction 79261) -> (junction 79260)
            (junction 79262) -> (junction 79261)
            (junction 79260) -> (junction 79263)
            (junction 79263) -> (junction 79264) [order 1] : [MOTION==1]
                | {MOTION=0;
                | UPDATE=true;}
            (junction 79264) -> Emergency.Doors.Closing0.Button_detection.Max_Min_assignment.Min_but1 [order 1] : [BUTTON_DOWN(1)]
            Emergency.Doors.Closing0.Button_detection.Max_Min_assignment.Min_but1 -> (junction 79265)
            (junction 79263) -> (junction 79269) [order 2]
            (junction 79264) -> (junction 79266) [order 2]
            (junction 79265) -> (junction 79267)
            (junction 79266) -> Emergency.Doors.Closing0.Button_detection.Max_Min_assignment.Min_but2 [order 1] : [BUTTON_DOWN(2)]
            Emergency.Doors.Closing0.Button_detection.Max_Min_assignment.Min_but2 -> (junction 79267)
            (junction 79266) -> Emergency.Doors.Closing0.Button_detection.Max_Min_assignment.Min_but3 [order 2]
            (junction 79267) -> (junction 79271)
            Emergency.Doors.Closing0.Button_detection.Max_Min_assignment.Min_but3 -> (junction 79270)
            (junction 79269) -> (junction 79268)
            (junction 79270) -> (junction 79269)
            (junction 79271) -> (junction 79270)
            (junction 79268) -> (junction 79273)
            Emergency.Doors.Closing0.Button_detection.Max_Min_assignment.MAX -> (junction 79272)
            (junction 79273) -> (junction 79274) [order 1] : [PUSHED]
            (junction 79274) -> (junction 79275) [order 1] : [not(BUT_TEMP==FLOOR) || not(MOTION==2)]
            (junction 79275) -> Emergency.Doors.Closing0.Button_detection.Max_Min_assignment.MAX [order 1] : [MAX_BUT<BUT_TEMP && not(UPDATE)]
            (junction 79272) -> (junction 79277)
            (junction 79273) -> (junction 79287) [order 2]
            (junction 79274) -> (junction 79280) [order 2]
            (junction 79275) -> (junction 79276) [order 2]
            (junction 79277) -> (junction 79276)
            (junction 79276) -> (junction 79278)
            (junction 79278) -> Emergency.Doors.Closing0.Button_detection.Max_Min_assignment.MIN [order 1] : [MIN_BUT>BUT_TEMP && not(UPDATE)]
            Emergency.Doors.Closing0.Button_detection.Max_Min_assignment.MIN -> (junction 79279)
            (junction 79278) -> (junction 79281) [order 2]
            (junction 79279) -> (junction 79282)
            (junction 79281) -> (junction 79280)
            (junction 79282) -> (junction 79281)
            (junction 79280) -> (junction 79283)
            (junction 79283) -> Emergency.Doors.Closing0.Button_detection.Max_Min_assignment.Updating_button_0 [order 1] : [MOTION==0]
            Emergency.Doors.Closing0.Button_detection.Max_Min_assignment.Updating_button_0 -> (junction 79284)
            (junction 79283) -> (junction 79285) [order 2]
            (junction 79284) -> (junction 79286)
            (junction 79285) -> Emergency.Doors.Closing0.Button_detection.Max_Min_assignment.Updating_button_1 [order 1] : [MOTION==1]
            Emergency.Doors.Closing0.Button_detection.Max_Min_assignment.Updating_button_1 -> (junction 79286)
            (junction 79285) -> (junction 79288) [order 2]
            (junction 79286) -> (junction 79289)
            (junction 79288) -> (junction 79287)
            (junction 79289) -> (junction 79288)
          state GoTo_PositionControl
            en:
            BUTTON=BUT_TEMP;
            FLAG=2;
          state Emergency
            en:
            FLAG_EMG=true;
            FLAG=4;
          state Timer_EME
            state Set_tmr
              en:
              Q_EME=true;
            state Counting
              en:
              ET_EME= ET_EME + 1;
              Q_EME=false;
            state Set
              en:
              IN_EME=true;
              PT_EME=3;
            (junction 79379) -> Emergency.Doors.Closing0.Button_detection.Timer_EME.Set_tmr [order 1] : [ET_EME==PT_EME]
            Emergency.Doors.Closing0.Button_detection.Timer_EME.Set_tmr -> (junction 79380)
            Emergency.Doors.Closing0.Button_detection.Timer_EME.Counting -> (junction 79379)
            (junction 79379) -> (junction 79380) [order 2]
            (default) -> Emergency.Doors.Closing0.Button_detection.Timer_EME.Set
            Emergency.Doors.Closing0.Button_detection.Timer_EME.Set -> (junction 79381)
            (junction 79381) -> Emergency.Doors.Closing0.Button_detection.Timer_EME.Counting [order 1] : [ET_EME<PT_EME]
            (junction 79381) -> (junction 79380) [order 2]
          state Not_Emergency
            en:
            IN_EME=false;
            ET_EME=0;
          state SwitchingOFF_LEDs
            en:
            LPD3=false;
            LPD2=false;
            LPS2=false;
            LPD1=false;
            LPS1=false;
            LPS0=false;
          (default) -> (junction 78980)
          (junction 78980) -> (junction 78981) [order 1] : [FLAG==1 && not(PUSHED)]
              | {BUTTON=FLOOR;
              | BUT_TEMP=BUTTON;
              | BUT_1=FLOOR;}
          (junction 78981) -> Emergency.Doors.Closing0.Button_detection.Timer_LL [order 1] : [not(FLAG_STOP)]
          Emergency.Doors.Closing0.Button_detection.Save_energy -> (junction 78982)
          Emergency.Doors.Closing0.Button_detection.Timer_LL -> Emergency.Doors.Closing0.Button_detection.Save_energy
          (junction 78981) -> (junction 78984) [order 2]
          (junction 78980) -> (junction 78983) [order 2]
          (junction 78982) -> (junction 78985)
          (junction 78984) -> (junction 78983)
          (junction 78985) -> (junction 78984)
          (junction 78983) -> Emergency.Doors.Closing0.Button_detection.BUTTON_CAR
          Emergency.Doors.Closing0.Button_detection.BUTTON_UP -> Emergency.Doors.Closing0.Button_detection.BUTTON_DOWN
          Emergency.Doors.Closing0.Button_detection.BUTTON_DOWN -> Emergency.Doors.Closing0.Button_detection.Max_Min_assignment
          Emergency.Doors.Closing0.Button_detection.Max_Min_assignment -> (junction 78986)
          Emergency.Doors.Closing0.Button_detection.BUTTON_CAR -> Emergency.Doors.Closing0.Button_detection.BUTTON_UP
          (junction 78986) -> (junction 78988)
          (junction 78988) -> (junction 78987)
          (junction 78987) -> (junction 78990)
          Emergency.Doors.Closing0.Button_detection.GoTo_PositionControl -> (junction 78989)
          (junction 78990) -> (junction 78991) [order 1] : [FLAG==1]
          (junction 78991) -> Emergency.Doors.Closing0.Button_detection.GoTo_PositionControl [order 1] : [PUSHED]
          (junction 78989) -> (junction 78993)
          (junction 78990) -> (junction 79001) [order 2]
          (junction 78991) -> (junction 78992) [order 2]
          (junction 78993) -> (junction 78992)
          (junction 78992) -> (junction 78995)
          Emergency.Doors.Closing0.Button_detection.Emergency -> (junction 78994)
          (junction 78995) -> Emergency.Doors.Closing0.Button_detection.Timer_EME [order 1] : [STOP]
              | {IN_LL=false; ET_LL=0;FLAG=1;}
          Emergency.Doors.Closing0.Button_detection.Timer_EME -> (junction 78996)
          (junction 78996) -> Emergency.Doors.Closing0.Button_detection.Emergency [order 1] : [Q_EME]
          (junction 78994) -> (junction 78998)
          (junction 78995) -> Emergency.Doors.Closing0.Button_detection.Not_Emergency [order 2]
          (junction 78996) -> (junction 78997) [order 2]
          (junction 78998) -> (junction 78997)
          (junction 78997) -> (junction 79000)
          Emergency.Doors.Closing0.Button_detection.Not_Emergency -> (junction 79000)
          Emergency.Doors.Closing0.Button_detection.SwitchingOFF_LEDs -> (junction 78999)
          (junction 79000) -> Emergency.Doors.Closing0.Button_detection.SwitchingOFF_LEDs [order 1] : [FLAG_STOP && FLAG==2]
          (junction 78999) -> (junction 79003)
          (junction 79000) -> (junction 79002) [order 2]
          (junction 79002) -> (junction 79001)
          (junction 79003) -> (junction 79002)
        state Extending
          en:
          EXTEND=true;
        state Stop_Closing
          en:
          CP0=false;
          FLAG_OD=false;
          OBS=false;
          ET_cl=0;
          IN_cl=false;
        state GoTo_PositionControl
          en: FLAG=2;
        state GoTo_BUttonDetection
          en:
          MOTION=2;
          MAX_BUT=0;
          MIN_BUT=3;
          PUSHED=false;
          FIRST_BUT=true;
          FLAG=1;
          UPDATE=false;
        state Closing1
          en:CP0=true;
        state Stop_Closing1
          en:CP0=false;
        Emergency.Doors.Closing0.Reset -> Emergency.Doors.Closing0.Timer_close
        (default) -> (junction 78891)
        (junction 78891) -> Emergency.Doors.Closing0.Reset [order 1] : [not(FLAG==0) && not(FLAG==4)]
        Emergency.Doors.Closing0.Timer_close -> (junction 78892)
        (junction 78892) -> Emergency.Doors.Closing0.Closing [order 1] : [not(PC0)]
        Emergency.Doors.Closing0.Button_detection -> (junction 78893)
        Emergency.Doors.Closing0.Closing -> Emergency.Doors.Closing0.Button_detection
        (junction 78891) -> (junction 78901) [order 2]
        (junction 78892) -> (junction 78894) [order 2]
        (junction 78893) -> (junction 78899)
        (junction 78894) -> Emergency.Doors.Closing0.Extending [order 1] : [BUTTON==FLOOR]
        (junction 78894) -> (junction 78896) [order 2]
        Emergency.Doors.Closing0.Extending -> (junction 78895)
        (junction 78895) -> (junction 78896)
        (junction 78896) -> Emergency.Doors.Closing0.Stop_Closing
        Emergency.Doors.Closing0.Stop_Closing -> (junction 78897)
        (junction 78897) -> Emergency.Doors.Closing0.GoTo_PositionControl [order 2]
        (junction 78897) -> Emergency.Doors.Closing0.GoTo_BUttonDetection [order 1] : [not(BUTTON_CAR(1) || BUTTON_CAR(2) || BUTTON_CAR(3) || BUTTON_CAR(4) || BUTTON_UP(1) || BUTTON_UP(2) || BUTTON_UP(3) || BUTTON_DOWN(2) || BUTTON_DOWN(3) || BUTTON_DOWN(4))]
        Emergency.Doors.Closing0.GoTo_PositionControl -> (junction 78898)
        Emergency.Doors.Closing0.GoTo_BUttonDetection -> (junction 78898)
        (junction 78898) -> (junction 78899)
        (junction 78899) -> (junction 78900)
        (junction 78900) -> (junction 78902)
        (junction 78901) -> Emergency.Doors.Closing0.Closing1 [order 1] : [not(PC0)]
        Emergency.Doors.Closing0.Closing1 -> (junction 78902)
        (junction 78901) -> Emergency.Doors.Closing0.Stop_Closing1 [order 2]
        Emergency.Doors.Closing0.Stop_Closing1 -> (junction 78902)
      state Closing1
        state Reset
          state Reset_0
            en:
            LPS0=false;
            BUTTON_CAR(1)=false;
            BUTTON_UP(1)=false;
          state Reset_1
            en:
            LPS1=false;
            LPD1=false;
            BUTTON_CAR(2)=false;
            BUTTON_UP(2)=false;
            BUTTON_DOWN(2)=false;
          state Reset_2
            en:
            LPS2=false;
            LPD2=false;
            BUTTON_CAR(3)=false;
            BUTTON_UP(3)=false;
            BUTTON_DOWN(3)=false;
          state Reset_3
            en:
            LPD3=false;
            BUTTON_CAR(4)=false;
            BUTTON_DOWN(4)=false;
          (default) -> (junction 80464)
          (junction 80464) -> Emergency.Doors.Closing1.Reset.Reset_0 [order 1] : [FLOOR==0]
          Emergency.Doors.Closing1.Reset.Reset_0 -> (junction 80465)
          (junction 80464) -> (junction 80466) [order 2]
          (junction 80465) -> (junction 80467)
          (junction 80466) -> Emergency.Doors.Closing1.Reset.Reset_1 [order 1] : [FLOOR==1]
          Emergency.Doors.Closing1.Reset.Reset_1 -> (junction 80467)
          (junction 80466) -> (junction 80468) [order 2]
          (junction 80467) -> (junction 80469)
          (junction 80468) -> Emergency.Doors.Closing1.Reset.Reset_2 [order 1] : [FLOOR==2]
          Emergency.Doors.Closing1.Reset.Reset_2 -> (junction 80469)
          (junction 80468) -> (junction 80470) [order 2]
          (junction 80469) -> (junction 80471)
          (junction 80470) -> Emergency.Doors.Closing1.Reset.Reset_3 [order 1] : [FLOOR==3]
          Emergency.Doors.Closing1.Reset.Reset_3 -> (junction 80471)
          (junction 80470) -> (junction 80472) [order 2]
          (junction 80471) -> (junction 80473)
          (junction 80473) -> (junction 80472)
        state Timer_close
          state Set_tmr
            en: Q_cl=true;
          state Set
            en:PT_cl=5;
            IN_cl=true;
          state Counting
            en:ET_cl = ET_cl + 1;
            Q_cl=false;
          (junction 80497) -> Emergency.Doors.Closing1.Timer_close.Set_tmr [order 1] : [ET_cl==PT_cl]
          Emergency.Doors.Closing1.Timer_close.Set_tmr -> (junction 80498)
          (default) -> Emergency.Doors.Closing1.Timer_close.Set
          Emergency.Doors.Closing1.Timer_close.Counting -> (junction 80497)
          (junction 80497) -> (junction 80498) [order 2]
          Emergency.Doors.Closing1.Timer_close.Set -> (junction 80499)
          (junction 80499) -> Emergency.Doors.Closing1.Timer_close.Counting [order 1] : [ET_cl<PT_cl]
          (junction 80499) -> (junction 80498) [order 2]
        state Closing
          en: CP1=Q_cl;
        state Button_detection
          state Save_energy
            en:
            LL=not(Q_LL);
          state Timer_LL
            state Set_tmr
              en:
              Q_LL=true;
            state Counting
              en:
              ET_LL= ET_LL + 1;
              Q_LL=false;
            state Set
              en:
              IN_LL=true;
              PT_LL=10;
            (junction 80581) -> Emergency.Doors.Closing1.Button_detection.Timer_LL.Set_tmr [order 1] : [ET_LL==PT_LL]
            Emergency.Doors.Closing1.Button_detection.Timer_LL.Set_tmr -> (junction 80582)
            Emergency.Doors.Closing1.Button_detection.Timer_LL.Counting -> (junction 80581)
            (junction 80581) -> (junction 80582) [order 2]
            (default) -> Emergency.Doors.Closing1.Button_detection.Timer_LL.Set
            Emergency.Doors.Closing1.Button_detection.Timer_LL.Set -> (junction 80583)
            (junction 80583) -> Emergency.Doors.Closing1.Button_detection.Timer_LL.Counting [order 1] : [ET_LL<PT_LL]
            (junction 80583) -> (junction 80582) [order 2]
          state BUTTON_DOWN
            state Button_DOWN_1
              en:
              BUTTON_DOWN(2)=true;
              BUT_TEMP=1;
              LPD1=true;
              PUSHED=true;
              UPDATE=false;
              IN_LL=false; ET_LL=0;
            state First_but_1
              en:
              BUT_1=BUT_TEMP;
              FIRST_BUT=false;
            state Button_DOWN_2
              en:
              BUTTON_DOWN(3)=true;
              BUT_TEMP=2;
              LPD2=true;
              PUSHED=true;
              UPDATE=false;
              IN_LL=false; ET_LL=0;
            state First_but_2
              en:
              BUT_1=BUT_TEMP;
              FIRST_BUT=false;
            state Button_DOWN_3
              en:
              BUTTON_DOWN(4)=true;
              BUT_TEMP=3;
              LPD3=true;
              PUSHED=true;
              UPDATE=false;
              IN_LL=false; ET_LL=0;
            state First_but_3
              en:
              BUT_1=BUT_TEMP;
              FIRST_BUT=false;
            (default) -> (junction 80596)
            (junction 80596) -> Emergency.Doors.Closing1.Button_detection.BUTTON_DOWN.Button_DOWN_1 [order 1] : [PD1]
            Emergency.Doors.Closing1.Button_detection.BUTTON_DOWN.Button_DOWN_1 -> (junction 80597)
            (junction 80597) -> Emergency.Doors.Closing1.Button_detection.BUTTON_DOWN.First_but_1 [order 1] : [FIRST_BUT && not(RPC1)]
            Emergency.Doors.Closing1.Button_detection.BUTTON_DOWN.First_but_1 -> (junction 80598)
            (junction 80596) -> (junction 80599) [order 2]
            (junction 80597) -> (junction 80600) [order 2]
            (junction 80598) -> (junction 80601)
            (junction 80600) -> (junction 80599)
            (junction 80601) -> (junction 80600)
            (junction 80599) -> (junction 80602)
            (junction 80602) -> Emergency.Doors.Closing1.Button_detection.BUTTON_DOWN.Button_DOWN_2 [order 1] : [PD2]
            Emergency.Doors.Closing1.Button_detection.BUTTON_DOWN.Button_DOWN_2 -> (junction 80603)
            (junction 80603) -> Emergency.Doors.Closing1.Button_detection.BUTTON_DOWN.First_but_2 [order 1] : [FIRST_BUT && not(RPC2)]
            Emergency.Doors.Closing1.Button_detection.BUTTON_DOWN.First_but_2 -> (junction 80604)
            (junction 80602) -> (junction 80605) [order 2]
            (junction 80603) -> (junction 80606) [order 2]
            (junction 80604) -> (junction 80607)
            (junction 80606) -> (junction 80605)
            (junction 80607) -> (junction 80606)
            (junction 80605) -> (junction 80608)
            (junction 80608) -> Emergency.Doors.Closing1.Button_detection.BUTTON_DOWN.Button_DOWN_3 [order 1] : [PD3]
            Emergency.Doors.Closing1.Button_detection.BUTTON_DOWN.Button_DOWN_3 -> (junction 80609)
            (junction 80609) -> Emergency.Doors.Closing1.Button_detection.BUTTON_DOWN.First_but_3 [order 1] : [FIRST_BUT && not(RPC3)]
            Emergency.Doors.Closing1.Button_detection.BUTTON_DOWN.First_but_3 -> (junction 80610)
            (junction 80608) -> (junction 80611) [order 2]
            (junction 80609) -> (junction 80612) [order 2]
            (junction 80610) -> (junction 80613)
            (junction 80612) -> (junction 80611)
            (junction 80613) -> (junction 80612)
          state BUTTON_CAR
            state Button_CAR_0
              en:
              BUTTON_CAR(1)=true;
              BUT_TEMP=0;
              LPC0=true;
              PUSHED=true;
              UPDATE=false;
              IN_LL=false; ET_LL=0;
            state First_but_0
              en:
              BUT_1=BUT_TEMP;
              FIRST_BUT=false;
            state Button_CAR_1
              en:
              BUTTON_CAR(2)=true;
              BUT_TEMP=1;
              LPC1=true;
              PUSHED=true;
              UPDATE=false;
              IN_LL=false; ET_LL=0;
            state First_but_1
              en:
              BUT_1=BUT_TEMP;
              FIRST_BUT=false;
            state Button_CAR_2
              en:
              BUTTON_CAR(3)=true;
              BUT_TEMP=2;
              LPC2=true;
              PUSHED=true;
              UPDATE=false;
              IN_LL=false; ET_LL=0;
            state First_but_2
              en:
              BUT_1=BUT_TEMP;
              FIRST_BUT=false;
            state Button_CAR_3
              en:
              BUTTON_CAR(4)=true;
              BUT_TEMP=3;
              LPC3=true;
              PUSHED=true;
              UPDATE=false;
              IN_LL=false; ET_LL=0;
            state First_but_3
              en:
              BUT_1=BUT_TEMP;
              FIRST_BUT=false;
            (default) -> (junction 80651)
            (junction 80651) -> Emergency.Doors.Closing1.Button_detection.BUTTON_CAR.Button_CAR_0 [order 1] : [P0]
            Emergency.Doors.Closing1.Button_detection.BUTTON_CAR.Button_CAR_0 -> (junction 80652)
            (junction 80652) -> Emergency.Doors.Closing1.Button_detection.BUTTON_CAR.First_but_0 [order 1] : [FIRST_BUT && not(RPC0)]
            Emergency.Doors.Closing1.Button_detection.BUTTON_CAR.First_but_0 -> (junction 80653)
            (junction 80651) -> (junction 80654) [order 2]
            (junction 80652) -> (junction 80655) [order 2]
            (junction 80653) -> (junction 80656)
            (junction 80655) -> (junction 80654)
            (junction 80656) -> (junction 80655)
            (junction 80654) -> (junction 80659)
            Emergency.Doors.Closing1.Button_detection.BUTTON_CAR.Button_CAR_1 -> (junction 80657)
            (junction 80657) -> Emergency.Doors.Closing1.Button_detection.BUTTON_CAR.First_but_1 [order 1] : [FIRST_BUT && not(RPC1)]
            Emergency.Doors.Closing1.Button_detection.BUTTON_CAR.First_but_1 -> (junction 80658)
            (junction 80657) -> (junction 80661) [order 2]
            (junction 80658) -> (junction 80662)
            (junction 80659) -> Emergency.Doors.Closing1.Button_detection.BUTTON_CAR.Button_CAR_1 [order 1] : [P1]
            (junction 80659) -> (junction 80660) [order 2]
            (junction 80661) -> (junction 80660)
            (junction 80662) -> (junction 80661)
            (junction 80660) -> (junction 80663)
            (junction 80663) -> Emergency.Doors.Closing1.Button_detection.BUTTON_CAR.Button_CAR_2 [order 1] : [P2]
            Emergency.Doors.Closing1.Button_detection.BUTTON_CAR.Button_CAR_2 -> (junction 80664)
            (junction 80664) -> Emergency.Doors.Closing1.Button_detection.BUTTON_CAR.First_but_2 [order 1] : [FIRST_BUT && not(RPC2)]
            Emergency.Doors.Closing1.Button_detection.BUTTON_CAR.First_but_2 -> (junction 80665)
            (junction 80663) -> (junction 80666) [order 2]
            (junction 80664) -> (junction 80667) [order 2]
            (junction 80665) -> (junction 80668)
            (junction 80667) -> (junction 80666)
            (junction 80668) -> (junction 80667)
            (junction 80666) -> (junction 80669)
            (junction 80669) -> Emergency.Doors.Closing1.Button_detection.BUTTON_CAR.Button_CAR_3 [order 1] : [P3]
            Emergency.Doors.Closing1.Button_detection.BUTTON_CAR.Button_CAR_3 -> (junction 80670)
            (junction 80670) -> Emergency.Doors.Closing1.Button_detection.BUTTON_CAR.First_but_3 [order 1] : [FIRST_BUT && not(RPC3)]
            Emergency.Doors.Closing1.Button_detection.BUTTON_CAR.First_but_3 -> (junction 80671)
            (junction 80669) -> (junction 80672) [order 2]
            (junction 80670) -> (junction 80673) [order 2]
            (junction 80671) -> (junction 80674)
            (junction 80673) -> (junction 80672)
            (junction 80674) -> (junction 80673)
          state BUTTON_UP
            state Button_UP_0
              en:
              BUTTON_UP(1)=true;
              BUT_TEMP=0;
              LPS0=true;
              PUSHED=true;
              UPDATE=false;
              IN_LL=false; ET_LL=0;
            state First_but_0
              en:
              BUT_1=BUT_TEMP;
              FIRST_BUT=false;
            state Button_UP_1
              en:
              BUTTON_UP(2)=true;
              BUT_TEMP=1;
              LPS1=true;
              PUSHED=true;
              UPDATE=false;
              IN_LL=false; ET_LL=0;
            state First_but_1
              en:
              BUT_1=BUT_TEMP;
              FIRST_BUT=false;
            state Button_UP_2
              en:
              BUTTON_UP(3)=true;
              BUT_TEMP=2;
              LPS2=true;
              PUSHED=true;
              UPDATE=false;
              IN_LL=false; ET_LL=0;
            state First_but_2
              en:
              BUT_1=BUT_TEMP;
              FIRST_BUT=false;
            (junction 80724) -> Emergency.Doors.Closing1.Button_detection.BUTTON_UP.Button_UP_0 [order 1] : [PS0]
            Emergency.Doors.Closing1.Button_detection.BUTTON_UP.Button_UP_0 -> (junction 80725)
            (junction 80725) -> Emergency.Doors.Closing1.Button_detection.BUTTON_UP.First_but_0 [order 1] : [FIRST_BUT && not(RPC0)]
            Emergency.Doors.Closing1.Button_detection.BUTTON_UP.First_but_0 -> (junction 80726)
            (default) -> (junction 80724)
            (junction 80724) -> (junction 80729) [order 2]
            (junction 80725) -> (junction 80727) [order 2]
            (junction 80726) -> (junction 80728)
            (junction 80728) -> (junction 80727)
            (junction 80727) -> (junction 80729)
            (junction 80729) -> (junction 80730)
            (junction 80730) -> Emergency.Doors.Closing1.Button_detection.BUTTON_UP.Button_UP_1 [order 1] : [PS1]
            Emergency.Doors.Closing1.Button_detection.BUTTON_UP.Button_UP_1 -> (junction 80731)
            (junction 80731) -> Emergency.Doors.Closing1.Button_detection.BUTTON_UP.First_but_1 [order 1] : [FIRST_BUT && not(RPC1)]
            Emergency.Doors.Closing1.Button_detection.BUTTON_UP.First_but_1 -> (junction 80732)
            (junction 80730) -> (junction 80733) [order 2]
            (junction 80731) -> (junction 80734) [order 2]
            (junction 80732) -> (junction 80735)
            (junction 80734) -> (junction 80733)
            (junction 80735) -> (junction 80734)
            (junction 80733) -> (junction 80737)
            Emergency.Doors.Closing1.Button_detection.BUTTON_UP.First_but_2 -> (junction 80736)
            (junction 80736) -> (junction 80741)
            (junction 80737) -> Emergency.Doors.Closing1.Button_detection.BUTTON_UP.Button_UP_2 [order 1] : [PS2]
            Emergency.Doors.Closing1.Button_detection.BUTTON_UP.Button_UP_2 -> (junction 80738)
            (junction 80738) -> Emergency.Doors.Closing1.Button_detection.BUTTON_UP.First_but_2 [order 1] : [FIRST_BUT && not(RPC2)]
            (junction 80737) -> (junction 80739) [order 2]
            (junction 80738) -> (junction 80740) [order 2]
            (junction 80740) -> (junction 80739)
            (junction 80741) -> (junction 80740)
          state Max_Min_assignment
            state Min_but
              en:
              BUTTON=MIN_BUT;
            state Max_but
              en:
              BUTTON=MAX_BUT;
            state First_but
              en:
              BUTTON=BUT_1;
            state Max_but1
              en:
              MAX_BUT=2;
            state Max_but2
              en:
              MAX_BUT=1;
            state Max_but3
              en:
              MAX_BUT=0;
            state Min_but1
              en:
              MIN_BUT=1;
            state Min_but2
              en:
              MIN_BUT=2;
            state Min_but3
              en:
              MIN_BUT=3;
            state MAX
              en:
              MAX_BUT=BUT_TEMP;
            state MIN
              en:
              MIN_BUT=BUT_TEMP;
            state Updating_button_0
              en:
              BUTTON=MAX_BUT;
            state Updating_button_1
              en:
              BUTTON=MIN_BUT;
            (junction 80779) -> Emergency.Doors.Closing1.Button_detection.Max_Min_assignment.Min_but [order 1] : [(MAX_BUT-FLOOR)>(FLOOR-MIN_BUT)]
            Emergency.Doors.Closing1.Button_detection.Max_Min_assignment.Min_but -> (junction 80780)
            (junction 80781) -> (junction 80779) [order 1] : [not(FLAG_STOP) && MOTION==2 && FLAG==3]
            (default) -> (junction 80781)
            (junction 80779) -> (junction 80782) [order 2]
            (junction 80780) -> (junction 80783)
            (junction 80781) -> (junction 80784) [order 2]
            (junction 80782) -> Emergency.Doors.Closing1.Button_detection.Max_Min_assignment.Max_but [order 1] : [(MAX_BUT-FLOOR)<(FLOOR-MIN_BUT)]
            Emergency.Doors.Closing1.Button_detection.Max_Min_assignment.Max_but -> (junction 80783)
            (junction 80782) -> Emergency.Doors.Closing1.Button_detection.Max_Min_assignment.First_but [order 2]
            (junction 80783) -> (junction 80786)
            Emergency.Doors.Closing1.Button_detection.Max_Min_assignment.First_but -> (junction 80785)
            (junction 80785) -> (junction 80784)
            (junction 80786) -> (junction 80785)
            (junction 80784) -> (junction 80787)
            (junction 80788) -> (junction 80789) [order 1] : [MOTION==0]
                | {MOTION=1;
                | UPDATE=true;}
            (junction 80789) -> Emergency.Doors.Closing1.Button_detection.Max_Min_assignment.Max_but1 [order 1] : [BUTTON_UP(2)]
            Emergency.Doors.Closing1.Button_detection.Max_Min_assignment.Max_but1 -> (junction 80790)
            (junction 80787) -> (junction 80788) [order 1] : [BUTTON==FLOOR && EXTEND]
                | {EXTEND=false;}
            (junction 80787) -> (junction 80801) [order 2]
            (junction 80788) -> (junction 80793) [order 2]
            (junction 80789) -> (junction 80791) [order 2]
            (junction 80790) -> (junction 80792)
            (junction 80791) -> Emergency.Doors.Closing1.Button_detection.Max_Min_assignment.Max_but2 [order 1] : [BUTTON_UP(1)]
            Emergency.Doors.Closing1.Button_detection.Max_Min_assignment.Max_but2 -> (junction 80792)
            (junction 80791) -> Emergency.Doors.Closing1.Button_detection.Max_Min_assignment.Max_but3 [order 2]
            (junction 80792) -> (junction 80795)
            Emergency.Doors.Closing1.Button_detection.Max_Min_assignment.Max_but3 -> (junction 80794)
            (junction 80794) -> (junction 80793)
            (junction 80795) -> (junction 80794)
            (junction 80793) -> (junction 80796)
            (junction 80796) -> (junction 80797) [order 1] : [MOTION==1]
                | {MOTION=0;
                | UPDATE=true;}
            (junction 80797) -> Emergency.Doors.Closing1.Button_detection.Max_Min_assignment.Min_but1 [order 1] : [BUTTON_DOWN(1)]
            Emergency.Doors.Closing1.Button_detection.Max_Min_assignment.Min_but1 -> (junction 80798)
            (junction 80796) -> (junction 80802) [order 2]
            (junction 80797) -> (junction 80799) [order 2]
            (junction 80798) -> (junction 80800)
            (junction 80799) -> Emergency.Doors.Closing1.Button_detection.Max_Min_assignment.Min_but2 [order 1] : [BUTTON_DOWN(2)]
            Emergency.Doors.Closing1.Button_detection.Max_Min_assignment.Min_but2 -> (junction 80800)
            (junction 80799) -> Emergency.Doors.Closing1.Button_detection.Max_Min_assignment.Min_but3 [order 2]
            (junction 80800) -> (junction 80804)
            Emergency.Doors.Closing1.Button_detection.Max_Min_assignment.Min_but3 -> (junction 80803)
            (junction 80802) -> (junction 80801)
            (junction 80803) -> (junction 80802)
            (junction 80804) -> (junction 80803)
            (junction 80801) -> (junction 80806)
            Emergency.Doors.Closing1.Button_detection.Max_Min_assignment.MAX -> (junction 80805)
            (junction 80806) -> (junction 80807) [order 1] : [PUSHED]
            (junction 80807) -> (junction 80808) [order 1] : [not(BUT_TEMP==FLOOR) || not(MOTION==2)]
            (junction 80808) -> Emergency.Doors.Closing1.Button_detection.Max_Min_assignment.MAX [order 1] : [MAX_BUT<BUT_TEMP && not(UPDATE)]
            (junction 80805) -> (junction 80810)
            (junction 80806) -> (junction 80820) [order 2]
            (junction 80807) -> (junction 80813) [order 2]
            (junction 80808) -> (junction 80809) [order 2]
            (junction 80810) -> (junction 80809)
            (junction 80809) -> (junction 80811)
            (junction 80811) -> Emergency.Doors.Closing1.Button_detection.Max_Min_assignment.MIN [order 1] : [MIN_BUT>BUT_TEMP && not(UPDATE)]
            Emergency.Doors.Closing1.Button_detection.Max_Min_assignment.MIN -> (junction 80812)
            (junction 80811) -> (junction 80814) [order 2]
            (junction 80812) -> (junction 80815)
            (junction 80814) -> (junction 80813)
            (junction 80815) -> (junction 80814)
            (junction 80813) -> (junction 80816)
            (junction 80816) -> Emergency.Doors.Closing1.Button_detection.Max_Min_assignment.Updating_button_0 [order 1] : [MOTION==0]
            Emergency.Doors.Closing1.Button_detection.Max_Min_assignment.Updating_button_0 -> (junction 80817)
            (junction 80816) -> (junction 80818) [order 2]
            (junction 80817) -> (junction 80819)
            (junction 80818) -> Emergency.Doors.Closing1.Button_detection.Max_Min_assignment.Updating_button_1 [order 1] : [MOTION==1]
            Emergency.Doors.Closing1.Button_detection.Max_Min_assignment.Updating_button_1 -> (junction 80819)
            (junction 80818) -> (junction 80821) [order 2]
            (junction 80819) -> (junction 80822)
            (junction 80821) -> (junction 80820)
            (junction 80822) -> (junction 80821)
          state GoTo_PositionControl
            en:
            BUTTON=BUT_TEMP;
            FLAG=2;
          state Emergency
            en:
            FLAG_EMG=true;
            FLAG=4;
          state Timer_EME
            state Set_tmr
              en:
              Q_EME=true;
            state Counting
              en:
              ET_EME= ET_EME + 1;
              Q_EME=false;
            state Set
              en:
              IN_EME=true;
              PT_EME=3;
            (junction 80912) -> Emergency.Doors.Closing1.Button_detection.Timer_EME.Set_tmr [order 1] : [ET_EME==PT_EME]
            Emergency.Doors.Closing1.Button_detection.Timer_EME.Set_tmr -> (junction 80913)
            Emergency.Doors.Closing1.Button_detection.Timer_EME.Counting -> (junction 80912)
            (junction 80912) -> (junction 80913) [order 2]
            (default) -> Emergency.Doors.Closing1.Button_detection.Timer_EME.Set
            Emergency.Doors.Closing1.Button_detection.Timer_EME.Set -> (junction 80914)
            (junction 80914) -> Emergency.Doors.Closing1.Button_detection.Timer_EME.Counting [order 1] : [ET_EME<PT_EME]
            (junction 80914) -> (junction 80913) [order 2]
          state Not_Emergency
            en:
            IN_EME=false;
            ET_EME=0;
          state SwitchingOFF_LEDs
            en:
            LPD3=false;
            LPD2=false;
            LPS2=false;
            LPD1=false;
            LPS1=false;
            LPS0=false;
          (default) -> (junction 80513)
          (junction 80513) -> (junction 80514) [order 1] : [FLAG==1 && not(PUSHED)]
              | {BUTTON=FLOOR;
              | BUT_TEMP=BUTTON;
              | BUT_1=FLOOR;}
          (junction 80514) -> Emergency.Doors.Closing1.Button_detection.Timer_LL [order 1] : [not(FLAG_STOP)]
          Emergency.Doors.Closing1.Button_detection.Save_energy -> (junction 80515)
          Emergency.Doors.Closing1.Button_detection.Timer_LL -> Emergency.Doors.Closing1.Button_detection.Save_energy
          (junction 80514) -> (junction 80517) [order 2]
          (junction 80513) -> (junction 80516) [order 2]
          (junction 80515) -> (junction 80518)
          (junction 80517) -> (junction 80516)
          (junction 80518) -> (junction 80517)
          (junction 80516) -> Emergency.Doors.Closing1.Button_detection.BUTTON_CAR
          Emergency.Doors.Closing1.Button_detection.BUTTON_UP -> Emergency.Doors.Closing1.Button_detection.BUTTON_DOWN
          Emergency.Doors.Closing1.Button_detection.BUTTON_DOWN -> Emergency.Doors.Closing1.Button_detection.Max_Min_assignment
          Emergency.Doors.Closing1.Button_detection.Max_Min_assignment -> (junction 80519)
          Emergency.Doors.Closing1.Button_detection.BUTTON_CAR -> Emergency.Doors.Closing1.Button_detection.BUTTON_UP
          (junction 80519) -> (junction 80521)
          (junction 80521) -> (junction 80520)
          (junction 80520) -> (junction 80523)
          Emergency.Doors.Closing1.Button_detection.GoTo_PositionControl -> (junction 80522)
          (junction 80523) -> (junction 80524) [order 1] : [FLAG==1]
          (junction 80524) -> Emergency.Doors.Closing1.Button_detection.GoTo_PositionControl [order 1] : [PUSHED]
          (junction 80522) -> (junction 80526)
          (junction 80523) -> (junction 80534) [order 2]
          (junction 80524) -> (junction 80525) [order 2]
          (junction 80526) -> (junction 80525)
          (junction 80525) -> (junction 80528)
          Emergency.Doors.Closing1.Button_detection.Emergency -> (junction 80527)
          (junction 80528) -> Emergency.Doors.Closing1.Button_detection.Timer_EME [order 1] : [STOP]
              | {IN_LL=false; ET_LL=0;FLAG=1;}
          Emergency.Doors.Closing1.Button_detection.Timer_EME -> (junction 80529)
          (junction 80529) -> Emergency.Doors.Closing1.Button_detection.Emergency [order 1] : [Q_EME]
          (junction 80527) -> (junction 80531)
          (junction 80528) -> Emergency.Doors.Closing1.Button_detection.Not_Emergency [order 2]
          (junction 80529) -> (junction 80530) [order 2]
          (junction 80531) -> (junction 80530)
          (junction 80530) -> (junction 80533)
          Emergency.Doors.Closing1.Button_detection.Not_Emergency -> (junction 80533)
          Emergency.Doors.Closing1.Button_detection.SwitchingOFF_LEDs -> (junction 80532)
          (junction 80533) -> Emergency.Doors.Closing1.Button_detection.SwitchingOFF_LEDs [order 1] : [FLAG_STOP && FLAG==2]
          (junction 80532) -> (junction 80536)
          (junction 80533) -> (junction 80535) [order 2]
          (junction 80535) -> (junction 80534)
          (junction 80536) -> (junction 80535)
        state Extending
          en:
          EXTEND=true;
        state Stop_Closing
          en:
          CP1=false;
          FLAG_OD=false;
          OBS=false;
          ET_cl=0;
          IN_cl=false;
        state GoTo_PositionControl
          en: FLAG=2;
        state GoTo_BUttonDetection
          en:
          MOTION=2;
          MAX_BUT=0;
          MIN_BUT=3;
          PUSHED=false;
          FIRST_BUT=true;
          FLAG=1;
          UPDATE=false;
        state Closing1
          en:CP1=true;
        state Stop_Closing1
          en:CP1=false;
        Emergency.Doors.Closing1.Reset -> Emergency.Doors.Closing1.Timer_close
        (default) -> (junction 80424)
        (junction 80424) -> Emergency.Doors.Closing1.Reset [order 1] : [not(FLAG==0) && not(FLAG==4)]
        Emergency.Doors.Closing1.Timer_close -> (junction 80425)
        (junction 80425) -> Emergency.Doors.Closing1.Closing [order 1] : [not(PC1)]
        Emergency.Doors.Closing1.Button_detection -> (junction 80426)
        Emergency.Doors.Closing1.Closing -> Emergency.Doors.Closing1.Button_detection
        (junction 80424) -> (junction 80434) [order 2]
        (junction 80425) -> (junction 80427) [order 2]
        (junction 80426) -> (junction 80432)
        (junction 80427) -> Emergency.Doors.Closing1.Extending [order 1] : [BUTTON==FLOOR]
        (junction 80427) -> (junction 80429) [order 2]
        Emergency.Doors.Closing1.Extending -> (junction 80428)
        (junction 80428) -> (junction 80429)
        (junction 80429) -> Emergency.Doors.Closing1.Stop_Closing
        Emergency.Doors.Closing1.Stop_Closing -> (junction 80430)
        (junction 80430) -> Emergency.Doors.Closing1.GoTo_PositionControl [order 2]
        (junction 80430) -> Emergency.Doors.Closing1.GoTo_BUttonDetection [order 1] : [not(BUTTON_CAR(1) || BUTTON_CAR(2) || BUTTON_CAR(3) || BUTTON_CAR(4) || BUTTON_UP(1) || BUTTON_UP(2) || BUTTON_UP(3) || BUTTON_DOWN(2) || BUTTON_DOWN(3) || BUTTON_DOWN(4))]
        Emergency.Doors.Closing1.GoTo_PositionControl -> (junction 80431)
        Emergency.Doors.Closing1.GoTo_BUttonDetection -> (junction 80431)
        (junction 80431) -> (junction 80432)
        (junction 80432) -> (junction 80433)
        (junction 80433) -> (junction 80435)
        (junction 80434) -> Emergency.Doors.Closing1.Closing1 [order 1] : [not(PC1)]
        Emergency.Doors.Closing1.Closing1 -> (junction 80435)
        (junction 80434) -> Emergency.Doors.Closing1.Stop_Closing1 [order 2]
        Emergency.Doors.Closing1.Stop_Closing1 -> (junction 80435)
      state Closing2
        state Reset
          state Reset_0
            en:
            LPS0=false;
            BUTTON_CAR(1)=false;
            BUTTON_UP(1)=false;
          state Reset_1
            en:
            LPS1=false;
            LPD1=false;
            BUTTON_CAR(2)=false;
            BUTTON_UP(2)=false;
            BUTTON_DOWN(2)=false;
          state Reset_2
            en:
            LPS2=false;
            LPD2=false;
            BUTTON_CAR(3)=false;
            BUTTON_UP(3)=false;
            BUTTON_DOWN(3)=false;
          state Reset_3
            en:
            LPD3=false;
            BUTTON_CAR(4)=false;
            BUTTON_DOWN(4)=false;
          (default) -> (junction 79442)
          (junction 79442) -> Emergency.Doors.Closing2.Reset.Reset_0 [order 1] : [FLOOR==0]
          Emergency.Doors.Closing2.Reset.Reset_0 -> (junction 79443)
          (junction 79442) -> (junction 79444) [order 2]
          (junction 79443) -> (junction 79445)
          (junction 79444) -> Emergency.Doors.Closing2.Reset.Reset_1 [order 1] : [FLOOR==1]
          Emergency.Doors.Closing2.Reset.Reset_1 -> (junction 79445)
          (junction 79444) -> (junction 79446) [order 2]
          (junction 79445) -> (junction 79447)
          (junction 79446) -> Emergency.Doors.Closing2.Reset.Reset_2 [order 1] : [FLOOR==2]
          Emergency.Doors.Closing2.Reset.Reset_2 -> (junction 79447)
          (junction 79446) -> (junction 79448) [order 2]
          (junction 79447) -> (junction 79449)
          (junction 79448) -> Emergency.Doors.Closing2.Reset.Reset_3 [order 1] : [FLOOR==3]
          Emergency.Doors.Closing2.Reset.Reset_3 -> (junction 79449)
          (junction 79448) -> (junction 79450) [order 2]
          (junction 79449) -> (junction 79451)
          (junction 79451) -> (junction 79450)
        state Timer_close
          state Set_tmr
            en: Q_cl=true;
          state Set
            en:PT_cl=5;
            IN_cl=true;
          state Counting
            en:ET_cl = ET_cl + 1;
            Q_cl=false;
          (junction 79475) -> Emergency.Doors.Closing2.Timer_close.Set_tmr [order 1] : [ET_cl==PT_cl]
          Emergency.Doors.Closing2.Timer_close.Set_tmr -> (junction 79476)
          (default) -> Emergency.Doors.Closing2.Timer_close.Set
          Emergency.Doors.Closing2.Timer_close.Counting -> (junction 79475)
          (junction 79475) -> (junction 79476) [order 2]
          Emergency.Doors.Closing2.Timer_close.Set -> (junction 79477)
          (junction 79477) -> Emergency.Doors.Closing2.Timer_close.Counting [order 1] : [ET_cl<PT_cl]
          (junction 79477) -> (junction 79476) [order 2]
        state Closing
          en: CP2=Q_cl;
        state Button_detection
          state Save_energy
            en:
            LL=not(Q_LL);
          state Timer_LL
            state Set_tmr
              en:
              Q_LL=true;
            state Counting
              en:
              ET_LL= ET_LL + 1;
              Q_LL=false;
            state Set
              en:
              IN_LL=true;
              PT_LL=10;
            (junction 79559) -> Emergency.Doors.Closing2.Button_detection.Timer_LL.Set_tmr [order 1] : [ET_LL==PT_LL]
            Emergency.Doors.Closing2.Button_detection.Timer_LL.Set_tmr -> (junction 79560)
            Emergency.Doors.Closing2.Button_detection.Timer_LL.Counting -> (junction 79559)
            (junction 79559) -> (junction 79560) [order 2]
            (default) -> Emergency.Doors.Closing2.Button_detection.Timer_LL.Set
            Emergency.Doors.Closing2.Button_detection.Timer_LL.Set -> (junction 79561)
            (junction 79561) -> Emergency.Doors.Closing2.Button_detection.Timer_LL.Counting [order 1] : [ET_LL<PT_LL]
            (junction 79561) -> (junction 79560) [order 2]
          state BUTTON_DOWN
            state Button_DOWN_1
              en:
              BUTTON_DOWN(2)=true;
              BUT_TEMP=1;
              LPD1=true;
              PUSHED=true;
              UPDATE=false;
              IN_LL=false; ET_LL=0;
            state First_but_1
              en:
              BUT_1=BUT_TEMP;
              FIRST_BUT=false;
            state Button_DOWN_2
              en:
              BUTTON_DOWN(3)=true;
              BUT_TEMP=2;
              LPD2=true;
              PUSHED=true;
              UPDATE=false;
              IN_LL=false; ET_LL=0;
            state First_but_2
              en:
              BUT_1=BUT_TEMP;
              FIRST_BUT=false;
            state Button_DOWN_3
              en:
              BUTTON_DOWN(4)=true;
              BUT_TEMP=3;
              LPD3=true;
              PUSHED=true;
              UPDATE=false;
              IN_LL=false; ET_LL=0;
